simulink model "ng_pv_dynamic_dbus_p_1_sm_ng"  (Simulink 8.8)
settings: Solver=ode4  StartTime=0.0  StopTime=inf  FixedStep=0.000125  RelTol=1e-3  EnableMultiTasking=on
PreLoadFcn:
  | Ts=125e-6;Core_Num = 0; np=1; nq=1; Vmin=.9;
PostLoadFcn:
  | Ts=125e-6;Core_Num = 0; np=1; nq=1; Vmin=.9;
InitFcn:
  | Ts=125e-6;Core_Num = 0; np=1; nq=1; Vmin=.9;
undefined symbols (not defined in the file or in its folder): another_event_name, DiscIntNeverNeededParam, I, j, Left, my_event_name, Right, type, V, X
libraries: powerlib x316, simulink_extras x78, powerlib_meascontrol x47, ssn_lib x9, opal_lib x5, powerlib_extras x3, simulink x3, artemis x1, rtio_opalrt_ml605ex1 x1, rtlab x1, rtio_spectracom x1
(part 2 of 11)

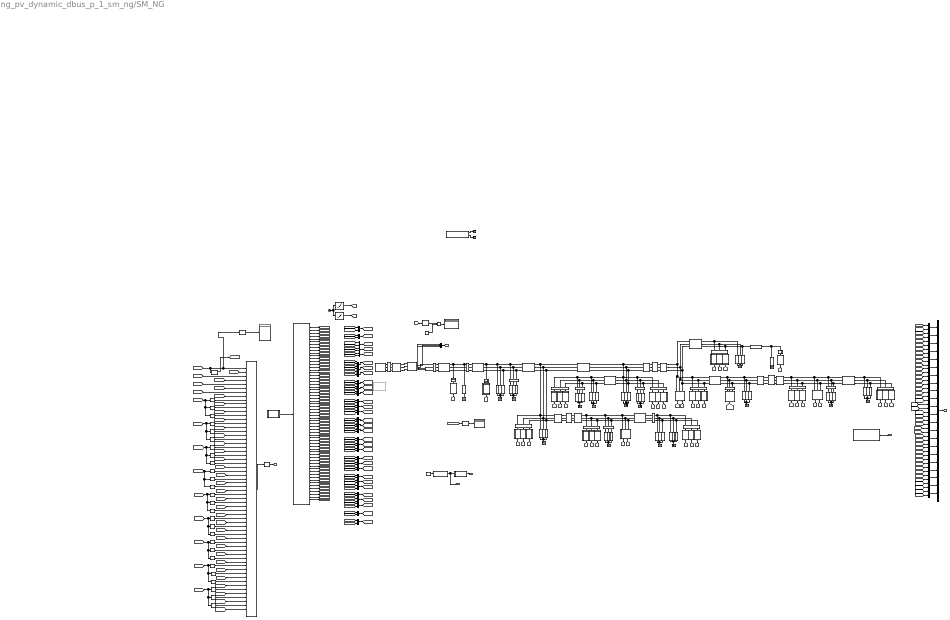
== system ng_pv_dynamic_dbus_p_1_sm_ng/SM_NG ==
  Bus Creator : BusCreator  Inputs=22
  Clock1 : Clock
  Constant : Constant  Value=13800/sqrt(3)
  Constant8 : Constant
  Demux1 : Demux  Outputs=62
  Display : Display
  Display1 : Display
  Divide : Product  Inputs=*/
  Dynamic Load BCDC1 : Subsystem
      mask Display:
      | plot(-45,-45,45,45,[0,9,18,24,29,30,29,24,18,9,0,-9,-18,-24,-29,-30,-29,-24,-18,-9,0]*.9,[30,29,24,18,9,0,-9,-18,-24,-29,-30,-29,-24,-18,-9,0,9,18,24,29,30]*.9)
      | plot([0,0,10,0,-10,0]*1.1,[15,-5,-5,-15,-5,-5]*1.1)
  Dynamic Load BCDC2 : Subsystem
      mask Display:
      | plot(-45,-45,45,45,[0,9,18,24,29,30,29,24,18,9,0,-9,-18,-24,-29,-30,-29,-24,-18,-9,0]*.9,[30,29,24,18,9,0,-9,-18,-24,-29,-30,-29,-24,-18,-9,0,9,18,24,29,30]*.9)
      | plot([0,0,10,0,-10,0]*1.1,[15,-5,-5,-15,-5,-5]*1.1)
  Dynamic Load BCDC3 : Subsystem
      mask Display:
      | plot(-45,-45,45,45,[0,9,18,24,29,30,29,24,18,9,0,-9,-18,-24,-29,-30,-29,-24,-18,-9,0]*.9,[30,29,24,18,9,0,-9,-18,-24,-29,-30,-29,-24,-18,-9,0,9,18,24,29,30]*.9)
      | plot([0,0,10,0,-10,0]*1.1,[15,-5,-5,-15,-5,-5]*1.1)
  Dynamic load measurement output1 : Display
  Ground{3,8,10,14,16,40,42..48,55,68..69} (16 alike) : powerlib/Elements/Ground  LConnTagsString=a
  IED1 : powerlib/Measurements/Three-Phase V-I Measurement  VoltageMeasurement=phase-to-ground  SetLabelV=on  LabelV=V_IED1  Vpu=off  VpuLL=off  CurrentMeasurement=yes  SetLabelI=on  LabelI=I_IED1  Ipu=off  Pbase=100e6  Vbase=500e3  OutputType=Complex  PhasorSimulation=off  PSBequivalent=0
  IED10 : Subsystem
      mask Display: %
  IED11 : powerlib/Measurements/Three-Phase V-I Measurement  VoltageMeasurement=phase-to-ground  SetLabelV=on  LabelV=V_IED11  Vpu=off  VpuLL=off  CurrentMeasurement=yes  SetLabelI=on  LabelI=I_IED11  Ipu=off  Pbase=100e6  Vbase=500e3  OutputType=Complex  PhasorSimulation=off  PSBequivalent=0
  IED12 : powerlib/Measurements/Three-Phase V-I Measurement  VoltageMeasurement=phase-to-ground  SetLabelV=on  LabelV=V_IED12  Vpu=off  VpuLL=off  CurrentMeasurement=yes  SetLabelI=on  LabelI=I_IED12  Ipu=off  Pbase=100e6  Vbase=500e3  OutputType=Complex  PhasorSimulation=off  PSBequivalent=0
  IED12A : powerlib/Measurements/Three-Phase V-I Measurement  VoltageMeasurement=phase-to-ground  SetLabelV=on  LabelV=V_IED12A  Vpu=off  VpuLL=off  CurrentMeasurement=yes  SetLabelI=on  LabelI=I_IED12A  Ipu=off  Pbase=100e6  Vbase=500e3  OutputType=Complex  PhasorSimulation=off  PSBequivalent=0
  IED13 : powerlib/Measurements/Three-Phase V-I Measurement  VoltageMeasurement=phase-to-ground  SetLabelV=on  LabelV=V_IED13  Vpu=off  VpuLL=off  CurrentMeasurement=yes  SetLabelI=on  LabelI=I_IED13  Ipu=off  Pbase=100e6  Vbase=500e3  OutputType=Complex  PhasorSimulation=off  PSBequivalent=0
  IED13A : powerlib/Measurements/Three-Phase V-I Measurement  VoltageMeasurement=phase-to-ground  SetLabelV=on  LabelV=V_IED13A  Vpu=off  VpuLL=off  CurrentMeasurement=yes  SetLabelI=on  LabelI=I_IED13A  Ipu=off  Pbase=100e6  Vbase=500e3  OutputType=Complex  PhasorSimulation=off  PSBequivalent=0
  IED14 : powerlib/Measurements/Three-Phase V-I Measurement  VoltageMeasurement=phase-to-ground  SetLabelV=on  LabelV=V_IED14  Vpu=off  VpuLL=off  CurrentMeasurement=yes  SetLabelI=on  LabelI=I_IED14  Ipu=off  Pbase=100e6  Vbase=500e3  OutputType=Complex  PhasorSimulation=off  PSBequivalent=0
  IED14A : Subsystem
      mask Display: %
  IED15 : powerlib/Measurements/Three-Phase V-I Measurement  VoltageMeasurement=phase-to-ground  SetLabelV=on  LabelV=V_IED15  Vpu=off  VpuLL=off  CurrentMeasurement=yes  SetLabelI=on  LabelI=I_IED15  Ipu=off  Pbase=100e6  Vbase=500e3  OutputType=Complex  PhasorSimulation=off  PSBequivalent=0
  IED2 : powerlib/Measurements/Three-Phase V-I Measurement  VoltageMeasurement=phase-to-ground  SetLabelV=on  LabelV=V_IED2  Vpu=off  VpuLL=off  CurrentMeasurement=yes  SetLabelI=on  LabelI=I_IED2  Ipu=off  Pbase=100e6  Vbase=500e3  OutputType=Complex  PhasorSimulation=off  PSBequivalent=0
  IED2A : powerlib/Measurements/Three-Phase V-I Measurement  VoltageMeasurement=phase-to-ground  SetLabelV=on  LabelV=V_IED2A  Vpu=off  VpuLL=off  CurrentMeasurement=yes  SetLabelI=on  LabelI=I_IED2A  Ipu=off  Pbase=100e6  Vbase=500e3  OutputType=Complex  PhasorSimulation=off  PSBequivalent=0
  IED3 : powerlib/Measurements/Three-Phase V-I Measurement  VoltageMeasurement=phase-to-ground  SetLabelV=on  LabelV=V_IED3  Vpu=off  VpuLL=off  CurrentMeasurement=yes  SetLabelI=on  LabelI=I_IED3  Ipu=off  Pbase=100e6  Vbase=500e3  OutputType=Complex  PhasorSimulation=off  PSBequivalent=0
  IED4 : powerlib/Measurements/Three-Phase V-I Measurement  VoltageMeasurement=phase-to-ground  SetLabelV=on  LabelV=V_IED4  Vpu=off  VpuLL=off  CurrentMeasurement=yes  SetLabelI=on  LabelI=I_IED4  Ipu=off  Pbase=100e6  Vbase=500e3  OutputType=Complex  PhasorSimulation=off  PSBequivalent=0
  IED5 : powerlib/Measurements/Three-Phase V-I Measurement  VoltageMeasurement=phase-to-ground  SetLabelV=on  LabelV=V_IED5  Vpu=off  VpuLL=off  CurrentMeasurement=yes  SetLabelI=on  LabelI=I_IED5  Ipu=off  Pbase=100e6  Vbase=500e3  OutputType=Complex  PhasorSimulation=off  PSBequivalent=0
  IED5A : powerlib/Measurements/Three-Phase V-I Measurement  VoltageMeasurement=phase-to-ground  SetLabelV=on  LabelV=V_IED5A  Vpu=off  VpuLL=off  CurrentMeasurement=yes  SetLabelI=on  LabelI=I_IED5A  Ipu=off  Pbase=100e6  Vbase=500e3  OutputType=Complex  PhasorSimulation=off  PSBequivalent=0
  IED6 : powerlib/Measurements/Three-Phase V-I Measurement  VoltageMeasurement=phase-to-ground  SetLabelV=on  LabelV=V_IED6  Vpu=off  VpuLL=off  CurrentMeasurement=yes  SetLabelI=on  LabelI=I_IED6  Ipu=off  Pbase=100e6  Vbase=500e3  OutputType=Complex  PhasorSimulation=off  PSBequivalent=0
  IED6A : powerlib/Measurements/Three-Phase V-I Measurement  VoltageMeasurement=phase-to-ground  SetLabelV=on  LabelV=V_IED6A  Vpu=off  VpuLL=off  CurrentMeasurement=yes  SetLabelI=on  LabelI=I_IED6A  Ipu=off  Pbase=100e6  Vbase=500e3  OutputType=Complex  PhasorSimulation=off  PSBequivalent=0
  IED7 : powerlib/Measurements/Three-Phase V-I Measurement  VoltageMeasurement=phase-to-ground  SetLabelV=on  LabelV=V_IED7  Vpu=off  VpuLL=off  CurrentMeasurement=yes  SetLabelI=on  LabelI=I_IED7  Ipu=off  Pbase=100e6  Vbase=500e3  OutputType=Complex  PhasorSimulation=off  PSBequivalent=0
  IED7A : Subsystem
      mask Display: %
  IED8 : powerlib/Measurements/Three-Phase V-I Measurement  VoltageMeasurement=phase-to-ground  SetLabelV=on  LabelV=V_IED8  Vpu=off  VpuLL=off  CurrentMeasurement=yes  SetLabelI=on  LabelI=I_IED8  Ipu=off  Pbase=100e6  Vbase=500e3  OutputType=Complex  PhasorSimulation=off  PSBequivalent=0
  IED9 : powerlib/Measurements/Three-Phase V-I Measurement  VoltageMeasurement=phase-to-ground  SetLabelV=on  LabelV=V_IED9  Vpu=off  VpuLL=off  CurrentMeasurement=yes  SetLabelI=on  LabelI=I_IED9  Ipu=off  Pbase=100e6  Vbase=500e3  OutputType=Complex  PhasorSimulation=off  PSBequivalent=0
  Line1132 : powerlib/Elements/Three-Phase PI Section Line  LConnTagsString=a|b|c  RConnTagsString=A|B|C  Frequency=60  Resistances=[0.071333 1.193903]  Inductances=[0.000315639 0.00352311]  Capacitances=[1.83433E-07 2.8E-13]  Length=0.067056
  Line3 : powerlib/Elements/Three-Phase PI Section Line  Commented=on  LConnTagsString=a|b|c  RConnTagsString=A|B|C  Frequency=60  Resistances=[0.0339 0.0293]  Inductances=[1.0783 1.0436]/(2*pi()*60)  Capacitances=[1E-16 1E-16]  Length=1
  Line369 : powerlib/Elements/Three-Phase PI Section Line  LConnTagsString=a|b|c  RConnTagsString=A|B|C  Frequency=60  Resistances=[2.631377E-01 0.6660566]  Inductances=[0.001030059 0.003789301]  Capacitances=[1.0e-16 1.0e-16]  Length=5.012741
  Line405A : powerlib/Elements/Three-Phase PI Section Line  LConnTagsString=a|b|c  RConnTagsString=A|B|C  Frequency=60  Resistances=[0.1736172 0.5584416]  Inductances=[0.001078896 0.003407176]  Capacitances=[1E-16 1E-16]  Length=0.7351776/2
  Line405B : powerlib/Elements/Three-Phase PI Section Line  LConnTagsString=a|b|c  RConnTagsString=A|B|C  Frequency=60  Resistances=[0.1736172 0.5584416]  Inductances=[0.001078896 0.003407176]  Capacitances=[1E-16 1E-16]  Length=0.7351776/2
  Line425 : powerlib/Elements/Three-Phase PI Section Line  LConnTagsString=a|b|c  RConnTagsString=A|B|C  Frequency=60  Resistances=[0.2736189 0.6685028]  Inductances=[0.001062159 0.003997129]  Capacitances=[1.0e-16 1.0e-16]  Length=2.185111
  Line489 : powerlib/Elements/Three-Phase PI Section Line  LConnTagsString=a|b|c  RConnTagsString=A|B|C  Frequency=60  Resistances=[0.118123 0.5162969]  Inductances=[0.000848017 0.003875996]  Capacitances=[1.0e-16 1.0e-16]  Length=0.2593848
  Line491 : powerlib/Elements/Three-Phase PI Section Line  LConnTagsString=a|b|c  RConnTagsString=A|B|C  Frequency=60  Resistances=[0.1181207 0.5161311]  Inductances=[0.00084801 0.003875749]  Capacitances=[1.0e-16 1.0e-16]  Length=3.555187
  Line614 : powerlib/Elements/Pi Section Line  LConnTagsString=__new0  RConnTagsString=__new0  Frequency=60  Resistance=1.074502  Inductance=0.001854886  Capacitance=1e-18  Length=1.515161  PiSections=1  Measurements=None
      settings: AttributesFormatString=\n
  Line687 : powerlib/Elements/Three-Phase PI Section Line  LConnTagsString=a|b|c  RConnTagsString=A|B|C  Frequency=60  Resistances=[1.671830E-01 0.5617232]  Inductances=[0.000886022 0.00391557]  Capacitances=[1.0e-16 1.0e-16]  Length=0.745236
  Line718A : powerlib/Elements/Three-Phase PI Section Line  LConnTagsString=a|b|c  RConnTagsString=A|B|C  Frequency=60  Resistances=[1.670246E-01 0.5628342]  Inductances=[0.000882962 0.00392461]  Capacitances=[1.0e-16 1.0e-16]  Length=1.407871/2
  Line718B : powerlib/Elements/Three-Phase PI Section Line  LConnTagsString=a|b|c  RConnTagsString=A|B|C  Frequency=60  Resistances=[1.670246E-01 0.5628342]  Inductances=[0.000882962 0.00392461]  Capacitances=[1.0e-16 1.0e-16]  Length=1.407871/2
  Line775A : powerlib/Elements/Three-Phase PI Section Line  LConnTagsString=a|b|c  RConnTagsString=A|B|C  Frequency=60  Resistances=[0.167158 0.5649899]  Inductances=[0.000879297 0.003911286]  Capacitances=[1.0e-16 1.0e-16]  Length=1.061314/2
  Line775B : powerlib/Elements/Three-Phase PI Section Line  LConnTagsString=a|b|c  RConnTagsString=A|B|C  Frequency=60  Resistances=[0.167158 0.5649899]  Inductances=[0.000879297 0.003911286]  Capacitances=[1.0e-16 1.0e-16]  Length=1.061314/2
  Line777 : powerlib/Elements/Three-Phase PI Section Line  LConnTagsString=a|b|c  RConnTagsString=A|B|C  Frequency=60  Resistances=[0.1732583 0.5348146]  Inductances=[0.000986024 0.00348674]  Capacitances=[1E-16 1E-16]  Length=0.6230112
  Line809 : powerlib/Elements/Three-Phase PI Section Line  LConnTagsString=a|b|c  RConnTagsString=A|B|C  Frequency=60  Resistances=[0.2709616 0.6137313]  Inductances=[0.00111084 0.00345815]  Capacitances=[1.0e-16 1.0e-16]  Length=2.52923
  Line937 : powerlib/Elements/Three-Phase PI Section Line  LConnTagsString=a|b|c  RConnTagsString=A|B|C  Frequency=60  Resistances=[0.1181214 0.5162814]  Inductances=[0.000848012 0.003875967]  Capacitances=[1.0e-16 1.0e-16]  Length=3.339389
  Mux{,1..4,6..53} (53 alike) : Mux  Inputs=2
  Mux5 : Mux  Inputs=62
  Mux54 : Mux  Inputs=3
  OpCtrl ML605EX1 : rtio_opalrt_ml605ex1/OpCtrl ML605EX1  CtrlName='ML605EX1 Ctrl'  boardid=0  BitstreamFilename=ML605_2-EX-0029-2_2_6_61-32Aio_32DioSelectable-01-01.bin  numconfig=-1  mode=Master  externalClock=off  decimRtsi=0  calibIO=off  SampleTime=0  loadinport=-1
  OpMonitor : rtlab/Monitoring/OpMonitor  compute_time=off  real_step=off  idle_time=off  nb_overruns=on  user_time=off  user_name=my_event_name,another_event_name
  PLL (3ph)2 : powerlib_meascontrol/PLL/PLL (3ph)  Fmin=45  Par_Init=[0, 60]  ParK=[180, 3200, 1]  TcD=1e-4  MaxRateChangeFreq=12  FilterCutOffFreq=25  Ts=0  AGC=on
  PV11 : Subsystem
      mask Display:
      | plot(.2*[0 3.5 5 2 0], .2*[1 1 4.5 4.5 1])
      | plot(.2*[1.7 3.5], .2*[1 4.5])
      | plot(.2*[1.1 4.3], .2*[3 3])
      | plot(.2*[.6 3.9], .2*[2 2])
      | plot(.2*[1.7 4.7], .2*[3.9 3.9])
  RMS : powerlib_meascontrol/Measurements/RMS  TrueRMS=on  Freq=60  RMSInit=120  Ts=0
  RMS2 : powerlib_meascontrol/Measurements/RMS  TrueRMS=on  Freq=60  RMSInit=480  Ts=Ts
  RMS28 : powerlib_meascontrol/Measurements/RMS  TrueRMS=on  Freq=60  RMSInit=480  Ts=Ts
  RMS3 : powerlib_meascontrol/Measurements/RMS  TrueRMS=on  Freq=60  RMSInit=13.8e3/sqrt(3)  Ts=Ts
  Real Power : Lookup_n-D  NumberOfTableDimensions=1  BreakpointsForDimension1=|  Table=|  ExtrapMethod=Clip  RndMeth=Simplest  InputSameDT=on
      BreakpointsForDimension1=|
      | [0
      | 900
      | 1800
      | 2700
      | 3600
      | 4500
      | 5400
      | 6300
      | 7200
      | 8100
      | 9000
      | 9900
      | 10800
      | 11700
      | 12600
      | 13500
      | 14400
      | 15300
      | 16200
      | 17100
      | 18000
      | 18900
      | 19800
      | 20700
      | 21600
      | ]
      Table=|
      | [0.386455785
      | 0.35306969
      | 0.331026162
      | 0.30769857
      | 0.305344452
      | 0.311122953
      | 0.342154931
      | 0.435946389
      | 0.489666766
      | 0.534959927
      | 0.558308136
      | 0.579659692
      | 0.643062563
      | 0.611273703
      | 0.64816703
      | 0.579694179
      | 0.56936906
      | 0.534896062
      | 0.526366773
      | 0.521782301
      | 0.502521358
      | 0.511800972
      | 0.405864397
      | 0.369267928
      | 0.34401424]
  Real Power1 : Lookup_n-D  NumberOfTableDimensions=1  BreakpointsForDimension1=|  Table=|  ExtrapMethod=Clip  RndMeth=Simplest  InputSameDT=on
      BreakpointsForDimension1=|
      | [0
      | 900
      | 1800
      | 2700
      | 3600
      | 4500
      | 5400
      | 6300
      | 7200
      | 8100
      | 9000
      | 9900
      | 10800
      | 11700
      | 12600
      | 13500
      | 14400
      | 15300
      | 16200
      | 17100
      | 18000
      | 18900
      | 19800
      | 20700
      | 21600
      | ]
      Table=|
      | [0.386455785
      | 0.35306969
      | 0.331026162
      | 0.30769857
      | 0.305344452
      | 0.311122953
      | 0.342154931
      | 0.435946389
      | 0.489666766
      | 0.534959927
      | 0.558308136
      | 0.579659692
      | 0.643062563
      | 0.611273703
      | 0.64816703
      | 0.579694179
      | 0.56936906
      | 0.534896062
      | 0.526366773
      | 0.521782301
      | 0.502521358
      | 0.511800972
      | 0.405864397
      | 0.369267928
      | 0.34401424]
  SSN Interface Block (3ph) : ssn_lib/SSN Interface Block (3ph)  nb_phase=3  nb_port=2  p1_type=I-type(Left)  p2_type=I-type(Right)  p3_type=V-type(Left)  p4_type=V-type(Left)  p5_type=V-type(Left)  p6_type=V-type(Left)  p7_type=V-type(Left)  p8_type=V-type(Left)  p9_type=V-type(Left)  p10_type=V-type(Left)  p11_type=V-type(Left)  p12_type=V-type(Left)  p13_type=V-type(Left)  p14_type=V-type(Left)  p15_type=V-type(Left)  p16_type=V-type(Left)  I_port_shunt_resistance=1e9
  SSN Interface Block (3ph)1 : ssn_lib/SSN Interface Block (3ph)  nb_phase=3  nb_port=2  p1_type=I-type(Left)  p2_type=I-type(Right)  p3_type=V-type(Left)  p4_type=V-type(Left)  p5_type=V-type(Left)  p6_type=V-type(Left)  p7_type=V-type(Left)  p8_type=V-type(Left)  p9_type=V-type(Left)  p10_type=V-type(Left)  p11_type=V-type(Left)  p12_type=V-type(Left)  p13_type=V-type(Left)  p14_type=V-type(Left)  p15_type=V-type(Left)  p16_type=V-type(Left)  I_port_shunt_resistance=1e9
  SSN Interface Block (3ph)2 : ssn_lib/SSN Interface Block (3ph)  nb_phase=3  nb_port=2  p1_type=I-type(Left)  p2_type=I-type(Right)  p3_type=V-type(Left)  p4_type=V-type(Left)  p5_type=V-type(Left)  p6_type=V-type(Left)  p7_type=V-type(Left)  p8_type=V-type(Left)  p9_type=V-type(Left)  p10_type=V-type(Left)  p11_type=V-type(Left)  p12_type=V-type(Left)  p13_type=V-type(Left)  p14_type=V-type(Left)  p15_type=V-type(Left)  p16_type=V-type(Left)  I_port_shunt_resistance=1e9
  Selector{7,10,13,16,19,22,25,28,31} (9 alike) : Selector  InputPortWidth=3  IndexOptions=Index vector (dialog)  Indices=[2]  OutputSizes=1
  Selector{8,11,14,17,20,23,26,29,32} (9 alike) : Selector  InputPortWidth=3  IndexOptions=Index vector (dialog)  Indices=[3]  OutputSizes=1
  Selector{6,9,12,15,18,21,24,27,30} (9 alike) : Selector  InputPortWidth=3  IndexOptions=Index vector (dialog)  Indices=[1]  OutputSizes=1
  Series  Load100 : powerlib/Elements/Series RLC Load  LConnTagsString=a  RConnTagsString=__new0  NominalVoltage=7967.4337  NominalFrequency=60  ActivePower=95731.2873  InductivePower=45807.5351  CapacitivePower=0  Setx0=off  InitialVoltage=0  SetiL0=off  InitialCurrent=0  Measurements=None  LoadType=constant Z
  Series  Load22 : powerlib/Elements/Series RLC Load  LConnTagsString=a  RConnTagsString=__new0  NominalVoltage=7967.4337  NominalFrequency=60  ActivePower=331147.6000  InductivePower=210430.3000  CapacitivePower=0  Setx0=off  InitialVoltage=0  SetiL0=off  InitialCurrent=0  Measurements=None  LoadType=constant Z
  Series  Load23 : powerlib/Elements/Series RLC Load  LConnTagsString=a  RConnTagsString=__new0  NominalVoltage=7967.4337  NominalFrequency=60  ActivePower=241844.2000  InductivePower=147122.1000  CapacitivePower=0  Setx0=off  InitialVoltage=0  SetiL0=off  InitialCurrent=0  Measurements=None  LoadType=constant Z
  Series  Load24 : powerlib/Elements/Series RLC Load  LConnTagsString=a  RConnTagsString=__new0  NominalVoltage=7967.4337  NominalFrequency=60  ActivePower=195882.9000  InductivePower=92467.2000  CapacitivePower=0  Setx0=off  InitialVoltage=0  SetiL0=off  InitialCurrent=0  Measurements=None  LoadType=constant Z
  Series  Load28 : powerlib/Elements/Series RLC Load  LConnTagsString=a  RConnTagsString=__new0  NominalVoltage=7967.4337  NominalFrequency=60  ActivePower=4813.9386  InductivePower=3013.6069  CapacitivePower=0  Setx0=off  InitialVoltage=0  SetiL0=off  InitialCurrent=0  Measurements=None  LoadType=constant Z
  Series  Load{42,60,80..83,91..96} (12 alike) : powerlib/Elements/Series RLC Load  LConnTagsString=a  RConnTagsString=__new0  NominalVoltage=7970  NominalFrequency=60  ActivePower=0  InductivePower=0  CapacitivePower=600000/3  Setx0=off  InitialVoltage=0  SetiL0=off  InitialCurrent=0  Measurements=None  LoadType=constant Z
  Series  Load43 : powerlib/Elements/Series RLC Load  LConnTagsString=a  RConnTagsString=__new0  NominalVoltage=7967.4337  NominalFrequency=60  ActivePower=4551.0724  InductivePower=2264.2140  CapacitivePower=0  Setx0=off  InitialVoltage=0  SetiL0=off  InitialCurrent=0  Measurements=None  LoadType=constant Z
  Series  Load61 : powerlib/Elements/Series RLC Load  LConnTagsString=a  RConnTagsString=__new0  NominalVoltage=7967.4337  NominalFrequency=60  ActivePower=282693.5835  InductivePower=180806.3086  CapacitivePower=0  Setx0=off  InitialVoltage=0  SetiL0=off  InitialCurrent=0  Measurements=None  LoadType=constant Z
  Series  Load62 : powerlib/Elements/Series RLC Load  LConnTagsString=a  RConnTagsString=__new0  NominalVoltage=7967.4337  NominalFrequency=60  ActivePower=208215.9420  InductivePower=105579.1068  CapacitivePower=0  Setx0=off  InitialVoltage=0  SetiL0=off  InitialCurrent=0  Measurements=None  LoadType=constant Z
  Series  Load63 : powerlib/Elements/Series RLC Load  LConnTagsString=a  RConnTagsString=__new0  NominalVoltage=7967.4337  NominalFrequency=60  ActivePower=421137.8951  InductivePower=259530.0314  CapacitivePower=0  Setx0=off  InitialVoltage=0  SetiL0=off  InitialCurrent=0  Measurements=None  LoadType=constant Z
  Series  Load64 : powerlib/Elements/Series RLC Load  LConnTagsString=a  RConnTagsString=__new0  NominalVoltage=7967.4337  NominalFrequency=60  ActivePower=122799.6001  InductivePower=58366.8938  CapacitivePower=0  Setx0=off  InitialVoltage=0  SetiL0=off  InitialCurrent=0  Measurements=None  LoadType=constant Z
  Series  Load7 : powerlib/Elements/Series RLC Load  LConnTagsString=a  RConnTagsString=__new0  NominalVoltage=7967.4337  NominalFrequency=60  ActivePower=612731.0000  InductivePower=318097.6000  CapacitivePower=0  Setx0=off  InitialVoltage=0  SetiL0=off  InitialCurrent=0  Measurements=None  LoadType=constant Z
  Series  Load71 : powerlib/Elements/Series RLC Load  LConnTagsString=a  RConnTagsString=__new0  NominalVoltage=7967.4337  NominalFrequency=60  ActivePower=10751.6072  InductivePower=5034.6946  CapacitivePower=0  Setx0=off  InitialVoltage=0  SetiL0=off  InitialCurrent=0  Measurements=None  LoadType=constant Z
  Series  Load72 : powerlib/Elements/Series RLC Load  LConnTagsString=a  RConnTagsString=__new0  NominalVoltage=7967.4337  NominalFrequency=60  ActivePower=118772.0877  InductivePower=74481.4641  CapacitivePower=0  Setx0=off  InitialVoltage=0  SetiL0=off  InitialCurrent=0  Measurements=None  LoadType=constant Z
  Series  Load73 : powerlib/Elements/Series RLC Load  LConnTagsString=a  RConnTagsString=__new0  NominalVoltage=7967.4337  NominalFrequency=60  ActivePower=132738.7273  InductivePower=44254.9312  CapacitivePower=0  Setx0=off  InitialVoltage=0  SetiL0=off  InitialCurrent=0  Measurements=None  LoadType=constant Z
  Series  Load74 : powerlib/Elements/Series RLC Load  LConnTagsString=a  RConnTagsString=__new0  NominalVoltage=7967.4337  NominalFrequency=60  ActivePower=81396.3132  InductivePower=49692.8288  CapacitivePower=0  Setx0=off  InitialVoltage=0  SetiL0=off  InitialCurrent=0  Measurements=None  LoadType=constant Z
  Series  Load75 : powerlib/Elements/Series RLC Load  LConnTagsString=a  RConnTagsString=__new0  NominalVoltage=7967.4337  NominalFrequency=60  ActivePower=22321.0824  InductivePower=10622.5578  CapacitivePower=0  Setx0=off  InitialVoltage=0  SetiL0=off  InitialCurrent=0  Measurements=None  LoadType=constant Z
  Series  Load76 : powerlib/Elements/Series RLC Load  LConnTagsString=a  RConnTagsString=__new0  NominalVoltage=7967.4337  NominalFrequency=60  ActivePower=333509.6803  InductivePower=179550.2294  CapacitivePower=0  Setx0=off  InitialVoltage=0  SetiL0=off  InitialCurrent=0  Measurements=None  LoadType=constant Z
  Series  Load77 : powerlib/Elements/Series RLC Load  LConnTagsString=a  RConnTagsString=__new0  NominalVoltage=7967.4337  NominalFrequency=60  ActivePower=249017.5283  InductivePower=118318.2378  CapacitivePower=0  Setx0=off  InitialVoltage=0  SetiL0=off  InitialCurrent=0  Measurements=None  LoadType=constant Z
  Series  Load78 : powerlib/Elements/Series RLC Load  LConnTagsString=a  RConnTagsString=__new0  NominalVoltage=7967.4337  NominalFrequency=60  ActivePower=191185.4608  InductivePower=115039.6819  CapacitivePower=0  Setx0=off  InitialVoltage=0  SetiL0=off  InitialCurrent=0  Measurements=None  LoadType=constant Z
  Series  Load79 : powerlib/Elements/Series RLC Load  LConnTagsString=a  RConnTagsString=__new0  NominalVoltage=7967.4337  NominalFrequency=60  ActivePower=315752.0854  InductivePower=102715.4164  CapacitivePower=0  Setx0=off  InitialVoltage=0  SetiL0=off  InitialCurrent=0  Measurements=None  LoadType=constant Z
  Series  Load8 : powerlib/Elements/Series RLC Load  LConnTagsString=a  RConnTagsString=__new0  NominalVoltage=7967.4337  NominalFrequency=60  ActivePower=406958.6000  InductivePower=209692.6000  CapacitivePower=0  Setx0=off  InitialVoltage=0  SetiL0=off  InitialCurrent=0  Measurements=None  LoadType=constant Z
  Series  Load84 : powerlib/Elements/Series RLC Load  LConnTagsString=a  RConnTagsString=__new0  NominalVoltage=7970  NominalFrequency=60  ActivePower=0  InductivePower=0  CapacitivePower=1200000/3  Setx0=off  InitialVoltage=0  SetiL0=off  InitialCurrent=0  Measurements=None  LoadType=constant PQ
  Series  Load85 : powerlib/Elements/Series RLC Load  LConnTagsString=a  RConnTagsString=__new0  NominalVoltage=7970  NominalFrequency=60  ActivePower=0  InductivePower=0  CapacitivePower=1200000/3  Setx0=off  InitialVoltage=0  SetiL0=off  InitialCurrent=0  Measurements=None  LoadType=constant PQ
  Series  Load86 : powerlib/Elements/Series RLC Load  LConnTagsString=a  RConnTagsString=__new0  NominalVoltage=7967.4337  NominalFrequency=60  ActivePower=108322.5585  InductivePower=62208.1391  CapacitivePower=0  Setx0=off  InitialVoltage=0  SetiL0=off  InitialCurrent=0  Measurements=None  LoadType=constant Z
  Series  Load87 : powerlib/Elements/Series RLC Load  LConnTagsString=a  RConnTagsString=__new0  NominalVoltage=7970  NominalFrequency=60  ActivePower=0  InductivePower=0  CapacitivePower=1200000/3  Setx0=off  InitialVoltage=0  SetiL0=off  InitialCurrent=0  Measurements=None  LoadType=constant PQ
  Series  Load88 : powerlib/Elements/Series RLC Load  LConnTagsString=a  RConnTagsString=__new0  NominalVoltage=7970  NominalFrequency=60  ActivePower=0  InductivePower=0  CapacitivePower=900000/3  Setx0=off  InitialVoltage=0  SetiL0=off  InitialCurrent=0  Measurements=None  LoadType=constant Z
  Series  Load89 : powerlib/Elements/Series RLC Load  LConnTagsString=a  RConnTagsString=__new0  NominalVoltage=7970  NominalFrequency=60  ActivePower=0  InductivePower=0  CapacitivePower=900000/3  Setx0=off  InitialVoltage=0  SetiL0=off  InitialCurrent=0  Measurements=None  LoadType=constant Z
  Series  Load9 : powerlib/Elements/Series RLC Load  LConnTagsString=a  RConnTagsString=__new0  NominalVoltage=7967.4337  NominalFrequency=60  ActivePower=419138.0000  InductivePower=167037.2000  CapacitivePower=0  Setx0=off  InitialVoltage=0  SetiL0=off  InitialCurrent=0  Measurements=None  LoadType=constant Z
  Series  Load90 : powerlib/Elements/Series RLC Load  LConnTagsString=a  RConnTagsString=__new0  NominalVoltage=7970  NominalFrequency=60  ActivePower=0  InductivePower=0  CapacitivePower=900000/3  Setx0=off  InitialVoltage=0  SetiL0=off  InitialCurrent=0  Measurements=None  LoadType=constant Z
  Series  Load97 : powerlib/Elements/Series RLC Load  LConnTagsString=a  RConnTagsString=__new0  NominalVoltage=7967.4337  NominalFrequency=60  ActivePower=91473.9797  InductivePower=41476.5707  CapacitivePower=0  Setx0=off  InitialVoltage=0  SetiL0=off  InitialCurrent=0  Measurements=None  LoadType=constant Z
  Series  Load98 : powerlib/Elements/Series RLC Load  LConnTagsString=a  RConnTagsString=__new0  NominalVoltage=7967.4337  NominalFrequency=60  ActivePower=276895.7686  InductivePower=217638.0421  CapacitivePower=0  Setx0=off  InitialVoltage=0  SetiL0=off  InitialCurrent=0  Measurements=None  LoadType=constant Z
  Series  Load99 : powerlib/Elements/Series RLC Load  LConnTagsString=a  RConnTagsString=__new0  NominalVoltage=7967.4337  NominalFrequency=60  ActivePower=181389.9148  InductivePower=112840.1531  CapacitivePower=0  Setx0=off  InitialVoltage=0  SetiL0=off  InitialCurrent=0  Measurements=None  LoadType=constant Z
  Single-Phase Dynamic Load30 : Subsystem  DialogController=POWERSYS.PowerSysDialog  mask(Single-Phase Dynamic Load){NominalVoltage=|, ActiveReactivePowers=[-27219.200 432.132], PositiveSequence=[1 0], ExternalControl=on, NpNq=[np nq], TimeConstants=[0  0  0  0], MinimumVoltage=Vmin, LoadFlowParameters=[4,0,0,0,0]}
      mask NominalVoltage=|
      | [7967.43
      |  60]
      mask prompts: NominalVoltage "Nominal voltage and frequency  [Vn(Vrms) fn(Hz)]:"; ActiveReactivePowers "Active and reactive power at initial voltage [Po(W) Qo(var)]:"; PositiveSequence "Initial voltage Vo [Mag(pu) Phase (deg.)]:"; ExternalControl "External control of PQ"; NpNq "Parameters [ np  nq ]:"; TimeConstants "Time constants [Tp1 Tp2 Tq1 Tq2]  (s):"; MinimumVoltage "Minimum voltage Vmin (pu):"; LoadFlowParameters "Load Flow parameters"
      mask help:
      | Implements a single-phase dynamic load. Active  power P and reactive
      | power Q absorbed by the load vary as function of voltage V  according to the
      | following equations:
      |
      |   If V>Vmin, P and Q vary as follows:
      |        P = Po * (V/Vo)^np * (1+Tp1.s)/(1+Tp2.s)
      |        Q = Qo * (V/Vo)^nq * (1+Tq1.s)/(1+Tq2.s)
      |   if V<Vmin
      |      Same equations with np=nq=2 (constant impedance load)
      mask init:
      | Vmin=.1;
      | 
      | Vnom=7967.43; 
      | fnom=60;
      | P0=-27219.200;
      | Q0=432.132;
      | Mag_V0=1; 
      | Pha_V0=0;
      | V0_d=1;
      | V0_q=Mag_V0*sin(Pha_V0*pi/180);
      | np=1;
      | nq=1;
      | Tp1=0; 
      | Tp2=0; 
      | Tq1=0; 
      | Tq2=0;
      | Vbase=Vnom/sqrt(3)*sqrt(2);
      | % initial value of positive-sequence current I1
      | I1_init=(P0-j*Q0)/((V0_d-j*V0_q)*Vnom)/sqrt(3)*sqrt(2);
      | Mag_ia=abs(I1_init);
      | Phase_ia=angle(I1_init)*180/pi;
      | %
      | a=exp(j*2*pi/3);
      | power_initmask();
      mask Help: helpview(psbhelp)
      mask Callback ExternalControl: powericon('ThreePhaseDynamicLoadCback',gcb);
      mask Display:
      | plot(.2*[0 3.5 5 2 0], .2*[1 1 4.5 4.5 1])
      | 
      | plot(.2*[1.7 3.5], .2*[1 4.5])
      | 
      | plot(.2*[1.1 4.3], .2*[3 3])
      | 
      | plot(.2*[.6 3.9], .2*[2 2])
      | 
      | plot(.2*[1.7 4.7], .2*[3.9 3.9])
  Single-Phase Dynamic Load32 : Subsystem  DialogController=POWERSYS.PowerSysDialog  mask(Single-Phase Dynamic Load){NominalVoltage=|, ActiveReactivePowers=|, PositiveSequence=[1 0], ExternalControl=on, NpNq=[np nq], TimeConstants=[0  0  0  0], MinimumVoltage=Vmin, LoadFlowParameters=[4,0,0,0,0]}
      mask NominalVoltage=|
      | [7967.43
      | 60]
      mask ActiveReactivePowers=|
      | [-277874.000
      | -40319.906]
      mask prompts: NominalVoltage "Nominal voltage and frequency  [Vn(Vrms) fn(Hz)]:"; ActiveReactivePowers "Active and reactive power at initial voltage [Po(W) Qo(var)]:"; PositiveSequence "Initial voltage Vo [Mag(pu) Phase (deg.)]:"; ExternalControl "External control of PQ"; NpNq "Parameters [ np  nq ]:"; TimeConstants "Time constants [Tp1 Tp2 Tq1 Tq2]  (s):"; MinimumVoltage "Minimum voltage Vmin (pu):"; LoadFlowParameters "Load Flow parameters"
      mask help:
      | Implements a single-phase dynamic load. Active  power P and reactive
      | power Q absorbed by the load vary as function of voltage V  according to the
      | following equations:
      |
      |   If V>Vmin, P and Q vary as follows:
      |        P = Po * (V/Vo)^np * (1+Tp1.s)/(1+Tp2.s)
      |        Q = Qo * (V/Vo)^nq * (1+Tq1.s)/(1+Tq2.s)
      |   if V<Vmin
      |      Same equations with np=nq=2 (constant impedance load)
      mask init:
      | block = gcb;
      | Ts = 50e-6;
      | %
      | Vnom=NominalVoltage(1); 
      | fnom=NominalVoltage(2);
      | P0=ActiveReactivePowers(1);
      | Q0=ActiveReactivePowers(2);
      | Mag_V0=PositiveSequence(1); 
      | Pha_V0=PositiveSequence(2);
      | V0_d=Mag_V0*cos(Pha_V0*pi/180);
      | V0_q=Mag_V0*sin(Pha_V0*pi/180);
      | np=NpNq(1);
      | nq=NpNq(2);
      | Tp1=TimeConstants(1); 
      | Tp2=TimeConstants(2); 
      | Tq1=TimeConstants(3); 
      | Tq2=TimeConstants(4);
      | Vbase=Vnom/sqrt(3)*sqrt(2);
      | % initial value of positive-sequence current I1
      | I1_init=(P0-j*Q0)/((V0_d-j*V0_q)*Vnom)/sqrt(3)*sqrt(2);
      | Mag_ia=abs(I1_init);
      | Phase_ia=angle(I1_init)*180/pi;
      | %
      | Vmin=MinimumVoltage;
      | PQext=ExternalControl;
      | a=exp(j*2*pi/3);
      | power_initmask();
      mask Help: helpview(psbhelp)
      mask Callback ExternalControl: powericon('ThreePhaseDynamicLoadCback',gcb);
      mask Display:
      | plot(.2*[0 3.5 5 2 0], .2*[1 1 4.5 4.5 1])
      | plot(.2*[1.7 3.5], .2*[1 4.5])
      | plot(.2*[1.1 4.3], .2*[3 3])
      | plot(.2*[.6 3.9], .2*[2 2])
      | plot(.2*[1.7 4.7], .2*[3.9 3.9])
  Single-Phase Dynamic Load33 : Subsystem  DialogController=POWERSYS.PowerSysDialog  mask(Single-Phase Dynamic Load){NominalVoltage=|, ActiveReactivePowers=|, PositiveSequence=[1 0], ExternalControl=on, NpNq=[np nq], TimeConstants=[0  0  0  0], MinimumVoltage=Vmin, LoadFlowParameters=[4,0,0,0,0]}
      mask NominalVoltage=|
      | [7967.43
      | 60]
      mask ActiveReactivePowers=|
      | [-127775.000
      | 18152.596]
      mask prompts: NominalVoltage "Nominal voltage and frequency  [Vn(Vrms) fn(Hz)]:"; ActiveReactivePowers "Active and reactive power at initial voltage [Po(W) Qo(var)]:"; PositiveSequence "Initial voltage Vo [Mag(pu) Phase (deg.)]:"; ExternalControl "External control of PQ"; NpNq "Parameters [ np  nq ]:"; TimeConstants "Time constants [Tp1 Tp2 Tq1 Tq2]  (s):"; MinimumVoltage "Minimum voltage Vmin (pu):"; LoadFlowParameters "Load Flow parameters"
      mask help:
      | Implements a single-phase dynamic load. Active  power P and reactive
      | power Q absorbed by the load vary as function of voltage V  according to the
      | following equations:
      |
      |   If V>Vmin, P and Q vary as follows:
      |        P = Po * (V/Vo)^np * (1+Tp1.s)/(1+Tp2.s)
      |        Q = Qo * (V/Vo)^nq * (1+Tq1.s)/(1+Tq2.s)
      |   if V<Vmin
      |      Same equations with np=nq=2 (constant impedance load)
      mask init: same as ng_pv_dynamic_dbus_p_1_sm_ng/SM_NG/Single-Phase Dynamic Load32
      mask Help: helpview(psbhelp)
      mask Callback ExternalControl: powericon('ThreePhaseDynamicLoadCback',gcb);
      mask Display:
      | plot(.2*[0 3.5 5 2 0], .2*[1 1 4.5 4.5 1])
      | plot(.2*[1.7 3.5], .2*[1 4.5])
      | plot(.2*[1.1 4.3], .2*[3 3])
      | plot(.2*[.6 3.9], .2*[2 2])
      | plot(.2*[1.7 4.7], .2*[3.9 3.9])
  Single-Phase Dynamic Load34 : Subsystem  DialogController=POWERSYS.PowerSysDialog  mask(Single-Phase Dynamic Load){NominalVoltage=|, ActiveReactivePowers=[-26871.400 3823.801], PositiveSequence=[1 0], ExternalControl=on, NpNq=[np nq], TimeConstants=[0  0  0  0], MinimumVoltage=Vmin, LoadFlowParameters=[4,0,0,0,0]}
      mask NominalVoltage=|
      | [ 7967.43
      | 60 ]
      mask prompts: NominalVoltage "Nominal voltage and frequency  [Vn(Vrms) fn(Hz)]:"; ActiveReactivePowers "Active and reactive power at initial voltage [Po(W) Qo(var)]:"; PositiveSequence "Initial voltage Vo [Mag(pu) Phase (deg.)]:"; ExternalControl "External control of PQ"; NpNq "Parameters [ np  nq ]:"; TimeConstants "Time constants [Tp1 Tp2 Tq1 Tq2]  (s):"; MinimumVoltage "Minimum voltage Vmin (pu):"; LoadFlowParameters "Load Flow parameters"
      mask help:
      | Implements a single-phase dynamic load. Active  power P and reactive
      | power Q absorbed by the load vary as function of voltage V  according to the
      | following equations:
      |
      |   If V>Vmin, P and Q vary as follows:
      |        P = Po * (V/Vo)^np * (1+Tp1.s)/(1+Tp2.s)
      |        Q = Qo * (V/Vo)^nq * (1+Tq1.s)/(1+Tq2.s)
      |   if V<Vmin
      |      Same equations with np=nq=2 (constant impedance load)
      mask init: same as ng_pv_dynamic_dbus_p_1_sm_ng/SM_NG/Single-Phase Dynamic Load32
      mask Help: helpview(psbhelp)
      mask Callback ExternalControl: powericon('ThreePhaseDynamicLoadCback',gcb);
      mask Display:
      | plot(.2*[0 3.5 5 2 0], .2*[1 1 4.5 4.5 1])
      | plot(.2*[1.7 3.5], .2*[1 4.5])
      | plot(.2*[1.1 4.3], .2*[3 3])
      | plot(.2*[.6 3.9], .2*[2 2])
      | plot(.2*[1.7 4.7], .2*[3.9 3.9])
  Single-Phase Dynamic Load35 : Subsystem  DialogController=POWERSYS.PowerSysDialog  mask(Single-Phase Dynamic Load){NominalVoltage=|, ActiveReactivePowers=|, PositiveSequence=[1 0], ExternalControl=on, NpNq=[np nq], TimeConstants=[0  0  0  0], MinimumVoltage=Vmin, LoadFlowParameters=[4,0,0,0,0]}
      mask NominalVoltage=|
      | [7967.43
      | 60 ]
      mask ActiveReactivePowers=|
      | [-22406.000
      | 7310.955]
      mask prompts: NominalVoltage "Nominal voltage and frequency  [Vn(Vrms) fn(Hz)]:"; ActiveReactivePowers "Active and reactive power at initial voltage [Po(W) Qo(var)]:"; PositiveSequence "Initial voltage Vo [Mag(pu) Phase (deg.)]:"; ExternalControl "External control of PQ"; NpNq "Parameters [ np  nq ]:"; TimeConstants "Time constants [Tp1 Tp2 Tq1 Tq2]  (s):"; MinimumVoltage "Minimum voltage Vmin (pu):"; LoadFlowParameters "Load Flow parameters"
      mask help:
      | Implements a single-phase dynamic load. Active  power P and reactive
      | power Q absorbed by the load vary as function of voltage V  according to the
      | following equations:
      |
      |   If V>Vmin, P and Q vary as follows:
      |        P = Po * (V/Vo)^np * (1+Tp1.s)/(1+Tp2.s)
      |        Q = Qo * (V/Vo)^nq * (1+Tq1.s)/(1+Tq2.s)
      |   if V<Vmin
      |      Same equations with np=nq=2 (constant impedance load)
      mask init: same as ng_pv_dynamic_dbus_p_1_sm_ng/SM_NG/Single-Phase Dynamic Load32
      mask Help: helpview(psbhelp)
      mask Callback ExternalControl: powericon('ThreePhaseDynamicLoadCback',gcb);
      mask Display:
      | plot(.2*[0 3.5 5 2 0], .2*[1 1 4.5 4.5 1])
      | plot(.2*[1.7 3.5], .2*[1 4.5])
      | plot(.2*[1.1 4.3], .2*[3 3])
      | plot(.2*[.6 3.9], .2*[2 2])
      | plot(.2*[1.7 4.7], .2*[3.9 3.9])
  Single-Phase Dynamic Load36 : Subsystem  DialogController=POWERSYS.PowerSysDialog  mask(Single-Phase Dynamic Load){NominalVoltage=[7967.43 60 ], ActiveReactivePowers=|, PositiveSequence=[1 0], ExternalControl=on, NpNq=[np nq], TimeConstants=[0  0  0  0], MinimumVoltage=Vmin, LoadFlowParameters=[4,0,0,0,0]}
      mask ActiveReactivePowers=|
      | [-67722.700
      | -9601.870]
      mask prompts: NominalVoltage "Nominal voltage and frequency  [Vn(Vrms) fn(Hz)]:"; ActiveReactivePowers "Active and reactive power at initial voltage [Po(W) Qo(var)]:"; PositiveSequence "Initial voltage Vo [Mag(pu) Phase (deg.)]:"; ExternalControl "External control of PQ"; NpNq "Parameters [ np  nq ]:"; TimeConstants "Time constants [Tp1 Tp2 Tq1 Tq2]  (s):"; MinimumVoltage "Minimum voltage Vmin (pu):"; LoadFlowParameters "Load Flow parameters"
      mask help:
      | Implements a single-phase dynamic load. Active  power P and reactive
      | power Q absorbed by the load vary as function of voltage V  according to the
      | following equations:
      |
      |   If V>Vmin, P and Q vary as follows:
      |        P = Po * (V/Vo)^np * (1+Tp1.s)/(1+Tp2.s)
      |        Q = Qo * (V/Vo)^nq * (1+Tq1.s)/(1+Tq2.s)
      |   if V<Vmin
      |      Same equations with np=nq=2 (constant impedance load)
      mask init: same as ng_pv_dynamic_dbus_p_1_sm_ng/SM_NG/Single-Phase Dynamic Load32
      mask Help: helpview(psbhelp)
      mask Callback ExternalControl: powericon('ThreePhaseDynamicLoadCback',gcb);
      mask Display:
      | plot(.2*[0 3.5 5 2 0], .2*[1 1 4.5 4.5 1])
      | plot(.2*[1.7 3.5], .2*[1 4.5])
      | plot(.2*[1.1 4.3], .2*[3 3])
      | plot(.2*[.6 3.9], .2*[2 2])
      | plot(.2*[1.7 4.7], .2*[3.9 3.9])
  Single-Phase Dynamic Load37 : Subsystem  DialogController=POWERSYS.PowerSysDialog  mask(Single-Phase Dynamic Load){NominalVoltage=|, ActiveReactivePowers=[-57616.400 -8183.737], PositiveSequence=[1 0], ExternalControl=on, NpNq=[np nq], TimeConstants=[0  0  0  0], MinimumVoltage=Vmin, LoadFlowParameters=[4,0,0,0,0]}
      mask NominalVoltage=|
      | [7967.43
      |  60 ]
      mask prompts: NominalVoltage "Nominal voltage and frequency  [Vn(Vrms) fn(Hz)]:"; ActiveReactivePowers "Active and reactive power at initial voltage [Po(W) Qo(var)]:"; PositiveSequence "Initial voltage Vo [Mag(pu) Phase (deg.)]:"; ExternalControl "External control of PQ"; NpNq "Parameters [ np  nq ]:"; TimeConstants "Time constants [Tp1 Tp2 Tq1 Tq2]  (s):"; MinimumVoltage "Minimum voltage Vmin (pu):"; LoadFlowParameters "Load Flow parameters"
      mask help:
      | Implements a single-phase dynamic load. Active  power P and reactive
      | power Q absorbed by the load vary as function of voltage V  according to the
      | following equations:
      |
      |   If V>Vmin, P and Q vary as follows:
      |        P = Po * (V/Vo)^np * (1+Tp1.s)/(1+Tp2.s)
      |        Q = Qo * (V/Vo)^nq * (1+Tq1.s)/(1+Tq2.s)
      |   if V<Vmin
      |      Same equations with np=nq=2 (constant impedance load)
      mask init: same as ng_pv_dynamic_dbus_p_1_sm_ng/SM_NG/Single-Phase Dynamic Load32
      mask Help: helpview(psbhelp)
      mask Callback ExternalControl: powericon('ThreePhaseDynamicLoadCback',gcb);
      mask Display:
      | plot(.2*[0 3.5 5 2 0], .2*[1 1 4.5 4.5 1])
      | plot(.2*[1.7 3.5], .2*[1 4.5])
      | plot(.2*[1.1 4.3], .2*[3 3])
      | plot(.2*[.6 3.9], .2*[2 2])
      | plot(.2*[1.7 4.7], .2*[3.9 3.9])
  Single-Phase Dynamic Load38 : Subsystem  DialogController=POWERSYS.PowerSysDialog  mask(Single-Phase Dynamic Load){NominalVoltage=|, ActiveReactivePowers=[-13034.700 1861.143], PositiveSequence=[1 0], ExternalControl=on, NpNq=[np nq], TimeConstants=[0  0  0  0], MinimumVoltage=Vmin, LoadFlowParameters=[4,0,0,0,0]}
      mask NominalVoltage=|
      | [7967.43
      |  60 ]
      mask prompts: NominalVoltage "Nominal voltage and frequency  [Vn(Vrms) fn(Hz)]:"; ActiveReactivePowers "Active and reactive power at initial voltage [Po(W) Qo(var)]:"; PositiveSequence "Initial voltage Vo [Mag(pu) Phase (deg.)]:"; ExternalControl "External control of PQ"; NpNq "Parameters [ np  nq ]:"; TimeConstants "Time constants [Tp1 Tp2 Tq1 Tq2]  (s):"; MinimumVoltage "Minimum voltage Vmin (pu):"; LoadFlowParameters "Load Flow parameters"
      mask help:
      | Implements a single-phase dynamic load. Active  power P and reactive
      | power Q absorbed by the load vary as function of voltage V  according to the
      | following equations:
      |
      |   If V>Vmin, P and Q vary as follows:
      |        P = Po * (V/Vo)^np * (1+Tp1.s)/(1+Tp2.s)
      |        Q = Qo * (V/Vo)^nq * (1+Tq1.s)/(1+Tq2.s)
      |   if V<Vmin
      |      Same equations with np=nq=2 (constant impedance load)
      mask init: same as ng_pv_dynamic_dbus_p_1_sm_ng/SM_NG/Single-Phase Dynamic Load32
      mask Help: helpview(psbhelp)
      mask Callback ExternalControl: powericon('ThreePhaseDynamicLoadCback',gcb);
      mask Display:
      | plot(.2*[0 3.5 5 2 0], .2*[1 1 4.5 4.5 1])
      | plot(.2*[1.7 3.5], .2*[1 4.5])
      | plot(.2*[1.1 4.3], .2*[3 3])
      | plot(.2*[.6 3.9], .2*[2 2])
      | plot(.2*[1.7 4.7], .2*[3.9 3.9])
  Single-Phase Dynamic Load39 : Subsystem  DialogController=POWERSYS.PowerSysDialog  mask(Single-Phase Dynamic Load){NominalVoltage=|, ActiveReactivePowers=|, PositiveSequence=[1 0], ExternalControl=on, NpNq=[np nq], TimeConstants=[0  0  0  0], MinimumVoltage=Vmin, LoadFlowParameters=[4,0,0,0,0]}
      mask NominalVoltage=|
      | [7967.43
      |  60 ]
      mask ActiveReactivePowers=|
      | [-51807.900
      | -7365.107]
      mask prompts: NominalVoltage "Nominal voltage and frequency  [Vn(Vrms) fn(Hz)]:"; ActiveReactivePowers "Active and reactive power at initial voltage [Po(W) Qo(var)]:"; PositiveSequence "Initial voltage Vo [Mag(pu) Phase (deg.)]:"; ExternalControl "External control of PQ"; NpNq "Parameters [ np  nq ]:"; TimeConstants "Time constants [Tp1 Tp2 Tq1 Tq2]  (s):"; MinimumVoltage "Minimum voltage Vmin (pu):"; LoadFlowParameters "Load Flow parameters"
      mask help:
      | Implements a single-phase dynamic load. Active  power P and reactive
      | power Q absorbed by the load vary as function of voltage V  according to the
      | following equations:
      |
      |   If V>Vmin, P and Q vary as follows:
      |        P = Po * (V/Vo)^np * (1+Tp1.s)/(1+Tp2.s)
      |        Q = Qo * (V/Vo)^nq * (1+Tq1.s)/(1+Tq2.s)
      |   if V<Vmin
      |      Same equations with np=nq=2 (constant impedance load)
      mask init: same as ng_pv_dynamic_dbus_p_1_sm_ng/SM_NG/Single-Phase Dynamic Load32
      mask Help: helpview(psbhelp)
      mask Callback ExternalControl: powericon('ThreePhaseDynamicLoadCback',gcb);
      mask Display:
      | plot(.2*[0 3.5 5 2 0], .2*[1 1 4.5 4.5 1])
      | plot(.2*[1.7 3.5], .2*[1 4.5])
      | plot(.2*[1.1 4.3], .2*[3 3])
      | plot(.2*[.6 3.9], .2*[2 2])
      | plot(.2*[1.7 4.7], .2*[3.9 3.9])
  Single-Phase Dynamic Load40 : Subsystem  DialogController=POWERSYS.PowerSysDialog  mask(Single-Phase Dynamic Load){NominalVoltage=|, ActiveReactivePowers=|, PositiveSequence=[1 0], ExternalControl=on, NpNq=[np nq], TimeConstants=[0  0  0  0], MinimumVoltage=Vmin, LoadFlowParameters=[4,0,0,0,0]}
      mask NominalVoltage=|
      | [7967.43
      |  60 ]
      mask ActiveReactivePowers=|
      | [-18221.200
      | -2652.826]
      mask prompts: NominalVoltage "Nominal voltage and frequency  [Vn(Vrms) fn(Hz)]:"; ActiveReactivePowers "Active and reactive power at initial voltage [Po(W) Qo(var)]:"; PositiveSequence "Initial voltage Vo [Mag(pu) Phase (deg.)]:"; ExternalControl "External control of PQ"; NpNq "Parameters [ np  nq ]:"; TimeConstants "Time constants [Tp1 Tp2 Tq1 Tq2]  (s):"; MinimumVoltage "Minimum voltage Vmin (pu):"; LoadFlowParameters "Load Flow parameters"
      mask help:
      | Implements a single-phase dynamic load. Active  power P and reactive
      | power Q absorbed by the load vary as function of voltage V  according to the
      | following equations:
      |
      |   If V>Vmin, P and Q vary as follows:
      |        P = Po * (V/Vo)^np * (1+Tp1.s)/(1+Tp2.s)
      |        Q = Qo * (V/Vo)^nq * (1+Tq1.s)/(1+Tq2.s)
      |   if V<Vmin
      |      Same equations with np=nq=2 (constant impedance load)
      mask init: same as ng_pv_dynamic_dbus_p_1_sm_ng/SM_NG/Single-Phase Dynamic Load32
      mask Help: helpview(psbhelp)
      mask Callback ExternalControl: powericon('ThreePhaseDynamicLoadCback',gcb);
      mask Display:
      | plot(.2*[0 3.5 5 2 0], .2*[1 1 4.5 4.5 1])
      | plot(.2*[1.7 3.5], .2*[1 4.5])
      | plot(.2*[1.1 4.3], .2*[3 3])
      | plot(.2*[.6 3.9], .2*[2 2])
      | plot(.2*[1.7 4.7], .2*[3.9 3.9])
  Single-Phase Dynamic Load41 : Subsystem  DialogController=POWERSYS.PowerSysDialog  mask(Single-Phase Dynamic Load){NominalVoltage=|, ActiveReactivePowers=[-119379.000 21541.648], PositiveSequence=[1 0], ExternalControl=on, NpNq=[np nq], TimeConstants=[0  0  0  0], MinimumVoltage=Vmin, LoadFlowParameters=[4,0,0,0,0]}
      mask NominalVoltage=|
      | [7967.43
      |  60 ]
      mask prompts: NominalVoltage "Nominal voltage and frequency  [Vn(Vrms) fn(Hz)]:"; ActiveReactivePowers "Active and reactive power at initial voltage [Po(W) Qo(var)]:"; PositiveSequence "Initial voltage Vo [Mag(pu) Phase (deg.)]:"; ExternalControl "External control of PQ"; NpNq "Parameters [ np  nq ]:"; TimeConstants "Time constants [Tp1 Tp2 Tq1 Tq2]  (s):"; MinimumVoltage "Minimum voltage Vmin (pu):"; LoadFlowParameters "Load Flow parameters"
      mask help:
      | Implements a single-phase dynamic load. Active  power P and reactive
      | power Q absorbed by the load vary as function of voltage V  according to the
      | following equations:
      |
      |   If V>Vmin, P and Q vary as follows:
      |        P = Po * (V/Vo)^np * (1+Tp1.s)/(1+Tp2.s)
      |        Q = Qo * (V/Vo)^nq * (1+Tq1.s)/(1+Tq2.s)
      |   if V<Vmin
      |      Same equations with np=nq=2 (constant impedance load)
      mask init: same as ng_pv_dynamic_dbus_p_1_sm_ng/SM_NG/Single-Phase Dynamic Load32
      mask Help: helpview(psbhelp)
      mask Callback ExternalControl: powericon('ThreePhaseDynamicLoadCback',gcb);
      mask Display:
      | plot(.2*[0 3.5 5 2 0], .2*[1 1 4.5 4.5 1])
      | plot(.2*[1.7 3.5], .2*[1 4.5])
      | plot(.2*[1.1 4.3], .2*[3 3])
      | plot(.2*[.6 3.9], .2*[2 2])
      | plot(.2*[1.7 4.7], .2*[3.9 3.9])
  Single-Phase Dynamic Load42 : Subsystem  DialogController=POWERSYS.PowerSysDialog  mask(Single-Phase Dynamic Load){NominalVoltage=[7967.43 60 ], ActiveReactivePowers=[-29638.700  -4207.799], PositiveSequence=[1 0], ExternalControl=on, NpNq=[np nq], TimeConstants=[0  0  0  0], MinimumVoltage=Vmin, LoadFlowParameters=[4,0,0,0,0]}
      mask prompts: NominalVoltage "Nominal voltage and frequency  [Vn(Vrms) fn(Hz)]:"; ActiveReactivePowers "Active and reactive power at initial voltage [Po(W) Qo(var)]:"; PositiveSequence "Initial voltage Vo [Mag(pu) Phase (deg.)]:"; ExternalControl "External control of PQ"; NpNq "Parameters [ np  nq ]:"; TimeConstants "Time constants [Tp1 Tp2 Tq1 Tq2]  (s):"; MinimumVoltage "Minimum voltage Vmin (pu):"; LoadFlowParameters "Load Flow parameters"
      mask help:
      | Implements a single-phase dynamic load. Active  power P and reactive
      | power Q absorbed by the load vary as function of voltage V  according to the
      | following equations:
      |
      |   If V>Vmin, P and Q vary as follows:
      |        P = Po * (V/Vo)^np * (1+Tp1.s)/(1+Tp2.s)
      |        Q = Qo * (V/Vo)^nq * (1+Tq1.s)/(1+Tq2.s)
      |   if V<Vmin
      |      Same equations with np=nq=2 (constant impedance load)
      mask init: same as ng_pv_dynamic_dbus_p_1_sm_ng/SM_NG/Single-Phase Dynamic Load32
      mask Help: helpview(psbhelp)
      mask Callback ExternalControl: powericon('ThreePhaseDynamicLoadCback',gcb);
      mask Display:
      | plot(.2*[0 3.5 5 2 0], .2*[1 1 4.5 4.5 1])
      | 
      | plot(.2*[1.7 3.5], .2*[1 4.5])
      | 
      | plot(.2*[1.1 4.3], .2*[3 3])
      | 
      | plot(.2*[.6 3.9], .2*[2 2])
      | 
      | plot(.2*[1.7 4.7], .2*[3.9 3.9])
  Single-Phase Dynamic Load43 : Subsystem  DialogController=POWERSYS.PowerSysDialog  mask(Single-Phase Dynamic Load){NominalVoltage=|, ActiveReactivePowers=[-53874.300 10730.813], PositiveSequence=[1 0], ExternalControl=on, NpNq=[np nq], TimeConstants=[0  0  0  0], MinimumVoltage=Vmin, LoadFlowParameters=[4,0,0,0,0]}
      mask NominalVoltage=|
      | [7967.43
      |  60 ]
      mask prompts: NominalVoltage "Nominal voltage and frequency  [Vn(Vrms) fn(Hz)]:"; ActiveReactivePowers "Active and reactive power at initial voltage [Po(W) Qo(var)]:"; PositiveSequence "Initial voltage Vo [Mag(pu) Phase (deg.)]:"; ExternalControl "External control of PQ"; NpNq "Parameters [ np  nq ]:"; TimeConstants "Time constants [Tp1 Tp2 Tq1 Tq2]  (s):"; MinimumVoltage "Minimum voltage Vmin (pu):"; LoadFlowParameters "Load Flow parameters"
      mask help:
      | Implements a single-phase dynamic load. Active  power P and reactive
      | power Q absorbed by the load vary as function of voltage V  according to the
      | following equations:
      |
      |   If V>Vmin, P and Q vary as follows:
      |        P = Po * (V/Vo)^np * (1+Tp1.s)/(1+Tp2.s)
      |        Q = Qo * (V/Vo)^nq * (1+Tq1.s)/(1+Tq2.s)
      |   if V<Vmin
      |      Same equations with np=nq=2 (constant impedance load)
      mask init: same as ng_pv_dynamic_dbus_p_1_sm_ng/SM_NG/Single-Phase Dynamic Load32
      mask Help: helpview(psbhelp)
      mask Callback ExternalControl: powericon('ThreePhaseDynamicLoadCback',gcb);
      mask Display:
      | plot(.2*[0 3.5 5 2 0], .2*[1 1 4.5 4.5 1])
      | plot(.2*[1.7 3.5], .2*[1 4.5])
      | plot(.2*[1.1 4.3], .2*[3 3])
      | plot(.2*[.6 3.9], .2*[2 2])
      | plot(.2*[1.7 4.7], .2*[3.9 3.9])
  Single-Phase Dynamic Load44 : Subsystem  DialogController=POWERSYS.PowerSysDialog  mask(Single-Phase Dynamic Load){NominalVoltage=|, ActiveReactivePowers=[-44033.300 -6802.859], PositiveSequence=[1 0], ExternalControl=on, NpNq=[np nq], TimeConstants=[0  0  0  0], MinimumVoltage=Vmin, LoadFlowParameters=[4,0,0,0,0]}
      mask NominalVoltage=|
      | [7967.00
      |  60 ]
      mask prompts: NominalVoltage "Nominal voltage and frequency  [Vn(Vrms) fn(Hz)]:"; ActiveReactivePowers "Active and reactive power at initial voltage [Po(W) Qo(var)]:"; PositiveSequence "Initial voltage Vo [Mag(pu) Phase (deg.)]:"; ExternalControl "External control of PQ"; NpNq "Parameters [ np  nq ]:"; TimeConstants "Time constants [Tp1 Tp2 Tq1 Tq2]  (s):"; MinimumVoltage "Minimum voltage Vmin (pu):"; LoadFlowParameters "Load Flow parameters"
      mask help:
      | Implements a single-phase dynamic load. Active  power P and reactive
      | power Q absorbed by the load vary as function of voltage V  according to the
      | following equations:
      |
      |   If V>Vmin, P and Q vary as follows:
      |        P = Po * (V/Vo)^np * (1+Tp1.s)/(1+Tp2.s)
      |        Q = Qo * (V/Vo)^nq * (1+Tq1.s)/(1+Tq2.s)
      |   if V<Vmin
      |      Same equations with np=nq=2 (constant impedance load)
      mask init: same as ng_pv_dynamic_dbus_p_1_sm_ng/SM_NG/Single-Phase Dynamic Load32
      mask Help: helpview(psbhelp)
      mask Callback ExternalControl: powericon('ThreePhaseDynamicLoadCback',gcb);
      mask Display:
      | plot(.2*[0 3.5 5 2 0], .2*[1 1 4.5 4.5 1])
      | plot(.2*[1.7 3.5], .2*[1 4.5])
      | plot(.2*[1.1 4.3], .2*[3 3])
      | plot(.2*[.6 3.9], .2*[2 2])
      | plot(.2*[1.7 4.7], .2*[3.9 3.9])
  Single-Phase Dynamic Load45 : Subsystem  DialogController=POWERSYS.PowerSysDialog  mask(Single-Phase Dynamic Load){NominalVoltage=|, ActiveReactivePowers=|, PositiveSequence=[1 0], ExternalControl=on, NpNq=[np nq], TimeConstants=[0  0  0  0], MinimumVoltage=Vmin, LoadFlowParameters=[4,0,0,0,0]}
      mask NominalVoltage=|
      | [7967.00
      |  60 ]
      mask ActiveReactivePowers=|
      | [-150415.000
      | -24442.388]
      mask prompts: NominalVoltage "Nominal voltage and frequency  [Vn(Vrms) fn(Hz)]:"; ActiveReactivePowers "Active and reactive power at initial voltage [Po(W) Qo(var)]:"; PositiveSequence "Initial voltage Vo [Mag(pu) Phase (deg.)]:"; ExternalControl "External control of PQ"; NpNq "Parameters [ np  nq ]:"; TimeConstants "Time constants [Tp1 Tp2 Tq1 Tq2]  (s):"; MinimumVoltage "Minimum voltage Vmin (pu):"; LoadFlowParameters "Load Flow parameters"
      mask help:
      | Implements a single-phase dynamic load. Active  power P and reactive
      | power Q absorbed by the load vary as function of voltage V  according to the
      | following equations:
      |
      |   If V>Vmin, P and Q vary as follows:
      |        P = Po * (V/Vo)^np * (1+Tp1.s)/(1+Tp2.s)
      |        Q = Qo * (V/Vo)^nq * (1+Tq1.s)/(1+Tq2.s)
      |   if V<Vmin
      |      Same equations with np=nq=2 (constant impedance load)
      mask init: same as ng_pv_dynamic_dbus_p_1_sm_ng/SM_NG/Single-Phase Dynamic Load32
      mask Help: helpview(psbhelp)
      mask Callback ExternalControl: powericon('ThreePhaseDynamicLoadCback',gcb);
      mask Display:
      | plot(.2*[0 3.5 5 2 0], .2*[1 1 4.5 4.5 1])
      | plot(.2*[1.7 3.5], .2*[1 4.5])
      | plot(.2*[1.1 4.3], .2*[3 3])
      | plot(.2*[.6 3.9], .2*[2 2])
      | plot(.2*[1.7 4.7], .2*[3.9 3.9])
  Single-Phase Dynamic Load46 : Subsystem  DialogController=POWERSYS.PowerSysDialog  mask(Single-Phase Dynamic Load){NominalVoltage=|, ActiveReactivePowers=|, PositiveSequence=[1 0], ExternalControl=on, NpNq=[np nq], TimeConstants=[0  0  0  0], MinimumVoltage=Vmin, LoadFlowParameters=[4,0,0,0,0]}
      mask NominalVoltage=|
      | [7967.00
      |  60 ]
      mask ActiveReactivePowers=|
      | [-21237.500
      | -6400.072]
      mask prompts: NominalVoltage "Nominal voltage and frequency  [Vn(Vrms) fn(Hz)]:"; ActiveReactivePowers "Active and reactive power at initial voltage [Po(W) Qo(var)]:"; PositiveSequence "Initial voltage Vo [Mag(pu) Phase (deg.)]:"; ExternalControl "External control of PQ"; NpNq "Parameters [ np  nq ]:"; TimeConstants "Time constants [Tp1 Tp2 Tq1 Tq2]  (s):"; MinimumVoltage "Minimum voltage Vmin (pu):"; LoadFlowParameters "Load Flow parameters"
      mask help:
      | Implements a single-phase dynamic load. Active  power P and reactive
      | power Q absorbed by the load vary as function of voltage V  according to the
      | following equations:
      |
      |   If V>Vmin, P and Q vary as follows:
      |        P = Po * (V/Vo)^np * (1+Tp1.s)/(1+Tp2.s)
      |        Q = Qo * (V/Vo)^nq * (1+Tq1.s)/(1+Tq2.s)
      |   if V<Vmin
      |      Same equations with np=nq=2 (constant impedance load)
      mask init: same as ng_pv_dynamic_dbus_p_1_sm_ng/SM_NG/Single-Phase Dynamic Load32
      mask Help: helpview(psbhelp)
      mask Callback ExternalControl: powericon('ThreePhaseDynamicLoadCback',gcb);
      mask Display:
      | plot(.2*[0 3.5 5 2 0], .2*[1 1 4.5 4.5 1])
      | plot(.2*[1.7 3.5], .2*[1 4.5])
      | plot(.2*[1.1 4.3], .2*[3 3])
      | plot(.2*[.6 3.9], .2*[2 2])
      | plot(.2*[1.7 4.7], .2*[3.9 3.9])
  Single-Phase Dynamic Load47 : Subsystem  DialogController=POWERSYS.PowerSysDialog  mask(Single-Phase Dynamic Load){NominalVoltage=|, ActiveReactivePowers=[-34508.300 4892.517], PositiveSequence=[1 0], ExternalControl=on, NpNq=[np nq], TimeConstants=[0  0  0  0], MinimumVoltage=Vmin, LoadFlowParameters=[4,0,0,0,0]}
      mask NominalVoltage=|
      | [7967.43
      |  60 ]
      mask prompts: NominalVoltage "Nominal voltage and frequency  [Vn(Vrms) fn(Hz)]:"; ActiveReactivePowers "Active and reactive power at initial voltage [Po(W) Qo(var)]:"; PositiveSequence "Initial voltage Vo [Mag(pu) Phase (deg.)]:"; ExternalControl "External control of PQ"; NpNq "Parameters [ np  nq ]:"; TimeConstants "Time constants [Tp1 Tp2 Tq1 Tq2]  (s):"; MinimumVoltage "Minimum voltage Vmin (pu):"; LoadFlowParameters "Load Flow parameters"
      mask help:
      | Implements a single-phase dynamic load. Active  power P and reactive
      | power Q absorbed by the load vary as function of voltage V  according to the
      | following equations:
      |
      |   If V>Vmin, P and Q vary as follows:
      |        P = Po * (V/Vo)^np * (1+Tp1.s)/(1+Tp2.s)
      |        Q = Qo * (V/Vo)^nq * (1+Tq1.s)/(1+Tq2.s)
      |   if V<Vmin
      |      Same equations with np=nq=2 (constant impedance load)
      mask init: same as ng_pv_dynamic_dbus_p_1_sm_ng/SM_NG/Single-Phase Dynamic Load32
      mask Help: helpview(psbhelp)
      mask Callback ExternalControl: powericon('ThreePhaseDynamicLoadCback',gcb);
      mask Display:
      | plot(.2*[0 3.5 5 2 0], .2*[1 1 4.5 4.5 1])
      | plot(.2*[1.7 3.5], .2*[1 4.5])
      | plot(.2*[1.1 4.3], .2*[3 3])
      | plot(.2*[.6 3.9], .2*[2 2])
      | plot(.2*[1.7 4.7], .2*[3.9 3.9])
  Single-Phase Dynamic Load48 : Subsystem  DialogController=POWERSYS.PowerSysDialog  mask(Single-Phase Dynamic Load){NominalVoltage=[ 7967.43 60 ], ActiveReactivePowers=|, PositiveSequence=[1 0], ExternalControl=on, NpNq=[np nq], TimeConstants=[0  0  0  0], MinimumVoltage=Vmin, LoadFlowParameters=[4,0,0,0,0]}
      mask ActiveReactivePowers=|
      | [-22450.700
      | 3182.886]
      mask prompts: NominalVoltage "Nominal voltage and frequency  [Vn(Vrms) fn(Hz)]:"; ActiveReactivePowers "Active and reactive power at initial voltage [Po(W) Qo(var)]:"; PositiveSequence "Initial voltage Vo [Mag(pu) Phase (deg.)]:"; ExternalControl "External control of PQ"; NpNq "Parameters [ np  nq ]:"; TimeConstants "Time constants [Tp1 Tp2 Tq1 Tq2]  (s):"; MinimumVoltage "Minimum voltage Vmin (pu):"; LoadFlowParameters "Load Flow parameters"
      mask help:
      | Implements a single-phase dynamic load. Active  power P and reactive
      | power Q absorbed by the load vary as function of voltage V  according to the
      | following equations:
      |
      |   If V>Vmin, P and Q vary as follows:
      |        P = Po * (V/Vo)^np * (1+Tp1.s)/(1+Tp2.s)
      |        Q = Qo * (V/Vo)^nq * (1+Tq1.s)/(1+Tq2.s)
      |   if V<Vmin
      |      Same equations with np=nq=2 (constant impedance load)
      mask init: same as ng_pv_dynamic_dbus_p_1_sm_ng/SM_NG/Single-Phase Dynamic Load32
      mask Help: helpview(psbhelp)
      mask Callback ExternalControl: powericon('ThreePhaseDynamicLoadCback',gcb);
      mask Display:
      | plot(.2*[0 3.5 5 2 0], .2*[1 1 4.5 4.5 1])
      | plot(.2*[1.7 3.5], .2*[1 4.5])
      | plot(.2*[1.1 4.3], .2*[3 3])
      | plot(.2*[.6 3.9], .2*[2 2])
      | plot(.2*[1.7 4.7], .2*[3.9 3.9])
  Single-Phase Dynamic Load49 : Subsystem  DialogController=POWERSYS.PowerSysDialog  mask(Single-Phase Dynamic Load){NominalVoltage=|, ActiveReactivePowers=|, PositiveSequence=[1 0], ExternalControl=on, NpNq=[np nq], TimeConstants=[0  0  0  0], MinimumVoltage=Vmin, LoadFlowParameters=[4,0,0,0,0]}
      mask NominalVoltage=|
      | [ 7967.43
      |  60 ]
      mask ActiveReactivePowers=|
      | [-9065.390
      | 1285.213]
      mask prompts: NominalVoltage "Nominal voltage and frequency  [Vn(Vrms) fn(Hz)]:"; ActiveReactivePowers "Active and reactive power at initial voltage [Po(W) Qo(var)]:"; PositiveSequence "Initial voltage Vo [Mag(pu) Phase (deg.)]:"; ExternalControl "External control of PQ"; NpNq "Parameters [ np  nq ]:"; TimeConstants "Time constants [Tp1 Tp2 Tq1 Tq2]  (s):"; MinimumVoltage "Minimum voltage Vmin (pu):"; LoadFlowParameters "Load Flow parameters"
      mask help:
      | Implements a single-phase dynamic load. Active  power P and reactive
      | power Q absorbed by the load vary as function of voltage V  according to the
      | following equations:
      |
      |   If V>Vmin, P and Q vary as follows:
      |        P = Po * (V/Vo)^np * (1+Tp1.s)/(1+Tp2.s)
      |        Q = Qo * (V/Vo)^nq * (1+Tq1.s)/(1+Tq2.s)
      |   if V<Vmin
      |      Same equations with np=nq=2 (constant impedance load)
      mask init: same as ng_pv_dynamic_dbus_p_1_sm_ng/SM_NG/Single-Phase Dynamic Load32
      mask Help: helpview(psbhelp)
      mask Callback ExternalControl: powericon('ThreePhaseDynamicLoadCback',gcb);
      mask Display:
      | plot(.2*[0 3.5 5 2 0], .2*[1 1 4.5 4.5 1])
      | plot(.2*[1.7 3.5], .2*[1 4.5])
      | plot(.2*[1.1 4.3], .2*[3 3])
      | plot(.2*[.6 3.9], .2*[2 2])
      | plot(.2*[1.7 4.7], .2*[3.9 3.9])
  Single-Phase Dynamic Load50 : Subsystem  DialogController=POWERSYS.PowerSysDialog  mask(Single-Phase Dynamic Load){NominalVoltage=[7967.43 60 ], ActiveReactivePowers=[-1001990.000 143475.169], PositiveSequence=[1 0], ExternalControl=on, NpNq=[np nq], TimeConstants=[0  0  0  0], MinimumVoltage=Vmin, LoadFlowParameters=[4,0,0,0,0]}
      mask prompts: NominalVoltage "Nominal voltage and frequency  [Vn(Vrms) fn(Hz)]:"; ActiveReactivePowers "Active and reactive power at initial voltage [Po(W) Qo(var)]:"; PositiveSequence "Initial voltage Vo [Mag(pu) Phase (deg.)]:"; ExternalControl "External control of PQ"; NpNq "Parameters [ np  nq ]:"; TimeConstants "Time constants [Tp1 Tp2 Tq1 Tq2]  (s):"; MinimumVoltage "Minimum voltage Vmin (pu):"; LoadFlowParameters "Load Flow parameters"
      mask help:
      | Implements a single-phase dynamic load. Active  power P and reactive
      | power Q absorbed by the load vary as function of voltage V  according to the
      | following equations:
      |
      |   If V>Vmin, P and Q vary as follows:
      |        P = Po * (V/Vo)^np * (1+Tp1.s)/(1+Tp2.s)
      |        Q = Qo * (V/Vo)^nq * (1+Tq1.s)/(1+Tq2.s)
      |   if V<Vmin
      |      Same equations with np=nq=2 (constant impedance load)
      mask init: same as ng_pv_dynamic_dbus_p_1_sm_ng/SM_NG/Single-Phase Dynamic Load32
      mask Help: helpview(psbhelp)
      mask Callback ExternalControl: powericon('ThreePhaseDynamicLoadCback',gcb);
      mask Display:
      | plot(.2*[0 3.5 5 2 0], .2*[1 1 4.5 4.5 1])
      | plot(.2*[1.7 3.5], .2*[1 4.5])
      | plot(.2*[1.1 4.3], .2*[3 3])
      | plot(.2*[.6 3.9], .2*[2 2])
      | plot(.2*[1.7 4.7], .2*[3.9 3.9])
  Single-Phase Dynamic Load51 : Subsystem  DialogController=POWERSYS.PowerSysDialog  mask(Single-Phase Dynamic Load){NominalVoltage=[7967.43 60 ], ActiveReactivePowers=|, PositiveSequence=[1 0], ExternalControl=on, NpNq=[np nq], TimeConstants=[0  0  0  0], MinimumVoltage=Vmin, LoadFlowParameters=[4,0,0,0,0]}
      mask ActiveReactivePowers=|
      | [-1018490.000
      | -144503.412]
      mask prompts: NominalVoltage "Nominal voltage and frequency  [Vn(Vrms) fn(Hz)]:"; ActiveReactivePowers "Active and reactive power at initial voltage [Po(W) Qo(var)]:"; PositiveSequence "Initial voltage Vo [Mag(pu) Phase (deg.)]:"; ExternalControl "External control of PQ"; NpNq "Parameters [ np  nq ]:"; TimeConstants "Time constants [Tp1 Tp2 Tq1 Tq2]  (s):"; MinimumVoltage "Minimum voltage Vmin (pu):"; LoadFlowParameters "Load Flow parameters"
      mask help:
      | Implements a single-phase dynamic load. Active  power P and reactive
      | power Q absorbed by the load vary as function of voltage V  according to the
      | following equations:
      |
      |   If V>Vmin, P and Q vary as follows:
      |        P = Po * (V/Vo)^np * (1+Tp1.s)/(1+Tp2.s)
      |        Q = Qo * (V/Vo)^nq * (1+Tq1.s)/(1+Tq2.s)
      |   if V<Vmin
      |      Same equations with np=nq=2 (constant impedance load)
      mask init: same as ng_pv_dynamic_dbus_p_1_sm_ng/SM_NG/Single-Phase Dynamic Load32
      mask Help: helpview(psbhelp)
      mask Callback ExternalControl: powericon('ThreePhaseDynamicLoadCback',gcb);
      mask Display:
      | plot(.2*[0 3.5 5 2 0], .2*[1 1 4.5 4.5 1])
      | plot(.2*[1.7 3.5], .2*[1 4.5])
      | plot(.2*[1.1 4.3], .2*[3 3])
      | plot(.2*[.6 3.9], .2*[2 2])
      | plot(.2*[1.7 4.7], .2*[3.9 3.9])
  Single-Phase Dynamic Load52 : Subsystem  DialogController=POWERSYS.PowerSysDialog  mask(Single-Phase Dynamic Load){NominalVoltage=[7967.43 60 ], ActiveReactivePowers=[-983676.000 139461.852], PositiveSequence=[1 0], ExternalControl=on, NpNq=[np nq], TimeConstants=[0  0  0  0], MinimumVoltage=Vmin, LoadFlowParameters=[4,0,0,0,0]}
      mask prompts: NominalVoltage "Nominal voltage and frequency  [Vn(Vrms) fn(Hz)]:"; ActiveReactivePowers "Active and reactive power at initial voltage [Po(W) Qo(var)]:"; PositiveSequence "Initial voltage Vo [Mag(pu) Phase (deg.)]:"; ExternalControl "External control of PQ"; NpNq "Parameters [ np  nq ]:"; TimeConstants "Time constants [Tp1 Tp2 Tq1 Tq2]  (s):"; MinimumVoltage "Minimum voltage Vmin (pu):"; LoadFlowParameters "Load Flow parameters"
      mask help:
      | Implements a single-phase dynamic load. Active  power P and reactive
      | power Q absorbed by the load vary as function of voltage V  according to the
      | following equations:
      |
      |   If V>Vmin, P and Q vary as follows:
      |        P = Po * (V/Vo)^np * (1+Tp1.s)/(1+Tp2.s)
      |        Q = Qo * (V/Vo)^nq * (1+Tq1.s)/(1+Tq2.s)
      |   if V<Vmin
      |      Same equations with np=nq=2 (constant impedance load)
      mask init: same as ng_pv_dynamic_dbus_p_1_sm_ng/SM_NG/Single-Phase Dynamic Load32
      mask Help: helpview(psbhelp)
      mask Callback ExternalControl: powericon('ThreePhaseDynamicLoadCback',gcb);
      mask Display:
      | plot(.2*[0 3.5 5 2 0], .2*[1 1 4.5 4.5 1])
      | plot(.2*[1.7 3.5], .2*[1 4.5])
      | plot(.2*[1.1 4.3], .2*[3 3])
      | plot(.2*[.6 3.9], .2*[2 2])
      | plot(.2*[1.7 4.7], .2*[3.9 3.9])
  Single-Phase Dynamic Load53 : Subsystem  DialogController=POWERSYS.PowerSysDialog  mask(Single-Phase Dynamic Load){NominalVoltage=[7967.43 60 ], ActiveReactivePowers=[-2219.570 -318.814], PositiveSequence=[1 0], ExternalControl=on, NpNq=[np nq], TimeConstants=[0  0  0  0], MinimumVoltage=Vmin, LoadFlowParameters=[4,0,0,0,0]}
      mask prompts: NominalVoltage "Nominal voltage and frequency  [Vn(Vrms) fn(Hz)]:"; ActiveReactivePowers "Active and reactive power at initial voltage [Po(W) Qo(var)]:"; PositiveSequence "Initial voltage Vo [Mag(pu) Phase (deg.)]:"; ExternalControl "External control of PQ"; NpNq "Parameters [ np  nq ]:"; TimeConstants "Time constants [Tp1 Tp2 Tq1 Tq2]  (s):"; MinimumVoltage "Minimum voltage Vmin (pu):"; LoadFlowParameters "Load Flow parameters"
      mask help:
      | Implements a single-phase dynamic load. Active  power P and reactive
      | power Q absorbed by the load vary as function of voltage V  according to the
      | following equations:
      |
      |   If V>Vmin, P and Q vary as follows:
      |        P = Po * (V/Vo)^np * (1+Tp1.s)/(1+Tp2.s)
      |        Q = Qo * (V/Vo)^nq * (1+Tq1.s)/(1+Tq2.s)
      |   if V<Vmin
      |      Same equations with np=nq=2 (constant impedance load)
      mask init: same as ng_pv_dynamic_dbus_p_1_sm_ng/SM_NG/Single-Phase Dynamic Load32
      mask Help: helpview(psbhelp)
      mask Callback ExternalControl: powericon('ThreePhaseDynamicLoadCback',gcb);
      mask Display:
      | plot(.2*[0 3.5 5 2 0], .2*[1 1 4.5 4.5 1])
      | plot(.2*[1.7 3.5], .2*[1 4.5])
      | plot(.2*[1.1 4.3], .2*[3 3])
      | plot(.2*[.6 3.9], .2*[2 2])
      | plot(.2*[1.7 4.7], .2*[3.9 3.9])
  Single-Phase Dynamic Load54 : Subsystem  DialogController=POWERSYS.PowerSysDialog  mask(Single-Phase Dynamic Load){NominalVoltage=|, ActiveReactivePowers=[-4738.140  2577.318], PositiveSequence=[1 0], ExternalControl=on, NpNq=[np nq], TimeConstants=[0  0  0  0], MinimumVoltage=Vmin, LoadFlowParameters=[4,0,0,0,0]}
      mask NominalVoltage=|
      | [7967.43
      | 60 ]
      mask prompts: NominalVoltage "Nominal voltage and frequency  [Vn(Vrms) fn(Hz)]:"; ActiveReactivePowers "Active and reactive power at initial voltage [Po(W) Qo(var)]:"; PositiveSequence "Initial voltage Vo [Mag(pu) Phase (deg.)]:"; ExternalControl "External control of PQ"; NpNq "Parameters [ np  nq ]:"; TimeConstants "Time constants [Tp1 Tp2 Tq1 Tq2]  (s):"; MinimumVoltage "Minimum voltage Vmin (pu):"; LoadFlowParameters "Load Flow parameters"
      mask help:
      | Implements a single-phase dynamic load. Active  power P and reactive
      | power Q absorbed by the load vary as function of voltage V  according to the
      | following equations:
      |
      |   If V>Vmin, P and Q vary as follows:
      |        P = Po * (V/Vo)^np * (1+Tp1.s)/(1+Tp2.s)
      |        Q = Qo * (V/Vo)^nq * (1+Tq1.s)/(1+Tq2.s)
      |   if V<Vmin
      |      Same equations with np=nq=2 (constant impedance load)
      mask init: same as ng_pv_dynamic_dbus_p_1_sm_ng/SM_NG/Single-Phase Dynamic Load32
      mask Help: helpview(psbhelp)
      mask Callback ExternalControl: powericon('ThreePhaseDynamicLoadCback',gcb);
      mask Display:
      | plot(.2*[0 3.5 5 2 0], .2*[1 1 4.5 4.5 1])
      | plot(.2*[1.7 3.5], .2*[1 4.5])
      | plot(.2*[1.1 4.3], .2*[3 3])
      | plot(.2*[.6 3.9], .2*[2 2])
      | plot(.2*[1.7 4.7], .2*[3.9 3.9])
  Single-Phase Dynamic Load55 : Subsystem  DialogController=POWERSYS.PowerSysDialog  mask(Single-Phase Dynamic Load){NominalVoltage=[7967.43 60 ], ActiveReactivePowers=[-92428.700 13104.122], PositiveSequence=[1 0], ExternalControl=on, NpNq=[np nq], TimeConstants=[0  0  0  0], MinimumVoltage=Vmin, LoadFlowParameters=[4,0,0,0,0]}
      mask prompts: NominalVoltage "Nominal voltage and frequency  [Vn(Vrms) fn(Hz)]:"; ActiveReactivePowers "Active and reactive power at initial voltage [Po(W) Qo(var)]:"; PositiveSequence "Initial voltage Vo [Mag(pu) Phase (deg.)]:"; ExternalControl "External control of PQ"; NpNq "Parameters [ np  nq ]:"; TimeConstants "Time constants [Tp1 Tp2 Tq1 Tq2]  (s):"; MinimumVoltage "Minimum voltage Vmin (pu):"; LoadFlowParameters "Load Flow parameters"
      mask help:
      | Implements a single-phase dynamic load. Active  power P and reactive
      | power Q absorbed by the load vary as function of voltage V  according to the
      | following equations:
      |
      |   If V>Vmin, P and Q vary as follows:
      |        P = Po * (V/Vo)^np * (1+Tp1.s)/(1+Tp2.s)
      |        Q = Qo * (V/Vo)^nq * (1+Tq1.s)/(1+Tq2.s)
      |   if V<Vmin
      |      Same equations with np=nq=2 (constant impedance load)
      mask init: same as ng_pv_dynamic_dbus_p_1_sm_ng/SM_NG/Single-Phase Dynamic Load32
      mask Help: helpview(psbhelp)
      mask Callback ExternalControl: powericon('ThreePhaseDynamicLoadCback',gcb);
      mask Display:
      | plot(.2*[0 3.5 5 2 0], .2*[1 1 4.5 4.5 1])
      | plot(.2*[1.7 3.5], .2*[1 4.5])
      | plot(.2*[1.1 4.3], .2*[3 3])
      | plot(.2*[.6 3.9], .2*[2 2])
      | plot(.2*[1.7 4.7], .2*[3.9 3.9])
  Single-Phase Dynamic Load56 : Subsystem  DialogController=POWERSYS.PowerSysDialog  mask(Single-Phase Dynamic Load){NominalVoltage=|, ActiveReactivePowers=[-58997.800 8411.427], PositiveSequence=[1 0], ExternalControl=on, NpNq=[np nq], TimeConstants=[0  0  0  0], MinimumVoltage=Vmin, LoadFlowParameters=[4,0,0,0,0]}
      mask NominalVoltage=|
      | [7967.43
      | 60]
      mask prompts: NominalVoltage "Nominal voltage and frequency  [Vn(Vrms) fn(Hz)]:"; ActiveReactivePowers "Active and reactive power at initial voltage [Po(W) Qo(var)]:"; PositiveSequence "Initial voltage Vo [Mag(pu) Phase (deg.)]:"; ExternalControl "External control of PQ"; NpNq "Parameters [ np  nq ]:"; TimeConstants "Time constants [Tp1 Tp2 Tq1 Tq2]  (s):"; MinimumVoltage "Minimum voltage Vmin (pu):"; LoadFlowParameters "Load Flow parameters"
      mask help:
      | Implements a single-phase dynamic load. Active  power P and reactive
      | power Q absorbed by the load vary as function of voltage V  according to the
      | following equations:
      |
      |   If V>Vmin, P and Q vary as follows:
      |        P = Po * (V/Vo)^np * (1+Tp1.s)/(1+Tp2.s)
      |        Q = Qo * (V/Vo)^nq * (1+Tq1.s)/(1+Tq2.s)
      |   if V<Vmin
      |      Same equations with np=nq=2 (constant impedance load)
      mask init: same as ng_pv_dynamic_dbus_p_1_sm_ng/SM_NG/Single-Phase Dynamic Load32
      mask Help: helpview(psbhelp)
      mask Callback ExternalControl: powericon('ThreePhaseDynamicLoadCback',gcb);
      mask Display:
      | plot(.2*[0 3.5 5 2 0], .2*[1 1 4.5 4.5 1])
      | plot(.2*[1.7 3.5], .2*[1 4.5])
      | plot(.2*[1.1 4.3], .2*[3 3])
      | plot(.2*[.6 3.9], .2*[2 2])
      | plot(.2*[1.7 4.7], .2*[3.9 3.9])
  Single-Phase Dynamic Load57 : Subsystem  DialogController=POWERSYS.PowerSysDialog  mask(Single-Phase Dynamic Load){NominalVoltage=[7967.43 60 ], ActiveReactivePowers=[-368952.000 56486.553], PositiveSequence=[1 0], ExternalControl=on, NpNq=[np nq], TimeConstants=[0  0  0  0], MinimumVoltage=Vmin, LoadFlowParameters=[4,0,0,0,0]}
      mask prompts: NominalVoltage "Nominal voltage and frequency  [Vn(Vrms) fn(Hz)]:"; ActiveReactivePowers "Active and reactive power at initial voltage [Po(W) Qo(var)]:"; PositiveSequence "Initial voltage Vo [Mag(pu) Phase (deg.)]:"; ExternalControl "External control of PQ"; NpNq "Parameters [ np  nq ]:"; TimeConstants "Time constants [Tp1 Tp2 Tq1 Tq2]  (s):"; MinimumVoltage "Minimum voltage Vmin (pu):"; LoadFlowParameters "Load Flow parameters"
      mask help:
      | Implements a single-phase dynamic load. Active  power P and reactive
      | power Q absorbed by the load vary as function of voltage V  according to the
      | following equations:
      |
      |   If V>Vmin, P and Q vary as follows:
      |        P = Po * (V/Vo)^np * (1+Tp1.s)/(1+Tp2.s)
      |        Q = Qo * (V/Vo)^nq * (1+Tq1.s)/(1+Tq2.s)
      |   if V<Vmin
      |      Same equations with np=nq=2 (constant impedance load)
      mask init: same as ng_pv_dynamic_dbus_p_1_sm_ng/SM_NG/Single-Phase Dynamic Load32
      mask Help: helpview(psbhelp)
      mask Callback ExternalControl: powericon('ThreePhaseDynamicLoadCback',gcb);
      mask Display:
      | plot(.2*[0 3.5 5 2 0], .2*[1 1 4.5 4.5 1])
      | plot(.2*[1.7 3.5], .2*[1 4.5])
      | plot(.2*[1.1 4.3], .2*[3 3])
      | plot(.2*[.6 3.9], .2*[2 2])
      | plot(.2*[1.7 4.7], .2*[3.9 3.9])
  Single-Phase Dynamic Load58 : Subsystem  DialogController=POWERSYS.PowerSysDialog  mask(Single-Phase Dynamic Load){NominalVoltage=|, ActiveReactivePowers=|, PositiveSequence=[1 0], ExternalControl=on, NpNq=[np nq], TimeConstants=[0  0  0  0], MinimumVoltage=Vmin, LoadFlowParameters=[4,0,0,0,0]}
      mask NominalVoltage=|
      | [7967.43
      | 60 ]
      mask ActiveReactivePowers=|
      | [-331064.000
      |  50291.023]
      mask prompts: NominalVoltage "Nominal voltage and frequency  [Vn(Vrms) fn(Hz)]:"; ActiveReactivePowers "Active and reactive power at initial voltage [Po(W) Qo(var)]:"; PositiveSequence "Initial voltage Vo [Mag(pu) Phase (deg.)]:"; ExternalControl "External control of PQ"; NpNq "Parameters [ np  nq ]:"; TimeConstants "Time constants [Tp1 Tp2 Tq1 Tq2]  (s):"; MinimumVoltage "Minimum voltage Vmin (pu):"; LoadFlowParameters "Load Flow parameters"
      mask help:
      | Implements a single-phase dynamic load. Active  power P and reactive
      | power Q absorbed by the load vary as function of voltage V  according to the
      | following equations:
      |
      |   If V>Vmin, P and Q vary as follows:
      |        P = Po * (V/Vo)^np * (1+Tp1.s)/(1+Tp2.s)
      |        Q = Qo * (V/Vo)^nq * (1+Tq1.s)/(1+Tq2.s)
      |   if V<Vmin
      |      Same equations with np=nq=2 (constant impedance load)
      mask init: same as ng_pv_dynamic_dbus_p_1_sm_ng/SM_NG/Single-Phase Dynamic Load32
      mask Help: helpview(psbhelp)
      mask Callback ExternalControl: powericon('ThreePhaseDynamicLoadCback',gcb);
      mask Display:
      | plot(.2*[0 3.5 5 2 0], .2*[1 1 4.5 4.5 1])
      | plot(.2*[1.7 3.5], .2*[1 4.5])
      | plot(.2*[1.1 4.3], .2*[3 3])
      | plot(.2*[.6 3.9], .2*[2 2])
      | plot(.2*[1.7 4.7], .2*[3.9 3.9])
  Single-Phase Dynamic Load59 : Subsystem  DialogController=POWERSYS.PowerSysDialog  mask(Single-Phase Dynamic Load){NominalVoltage=|, ActiveReactivePowers=|, PositiveSequence=[1 0], ExternalControl=on, NpNq=[np nq], TimeConstants=[0  0  0  0], MinimumVoltage=Vmin, LoadFlowParameters=[4,0,0,0,0]}
      mask NominalVoltage=|
      | [7967.43
      | 60 ]
      mask ActiveReactivePowers=|
      | [-340231.000
      | 51005.605]
      mask prompts: NominalVoltage "Nominal voltage and frequency  [Vn(Vrms) fn(Hz)]:"; ActiveReactivePowers "Active and reactive power at initial voltage [Po(W) Qo(var)]:"; PositiveSequence "Initial voltage Vo [Mag(pu) Phase (deg.)]:"; ExternalControl "External control of PQ"; NpNq "Parameters [ np  nq ]:"; TimeConstants "Time constants [Tp1 Tp2 Tq1 Tq2]  (s):"; MinimumVoltage "Minimum voltage Vmin (pu):"; LoadFlowParameters "Load Flow parameters"
      mask help:
      | Implements a single-phase dynamic load. Active  power P and reactive
      | power Q absorbed by the load vary as function of voltage V  according to the
      | following equations:
      |
      |   If V>Vmin, P and Q vary as follows:
      |        P = Po * (V/Vo)^np * (1+Tp1.s)/(1+Tp2.s)
      |        Q = Qo * (V/Vo)^nq * (1+Tq1.s)/(1+Tq2.s)
      |   if V<Vmin
      |      Same equations with np=nq=2 (constant impedance load)
      mask init: same as ng_pv_dynamic_dbus_p_1_sm_ng/SM_NG/Single-Phase Dynamic Load32
      mask Help: helpview(psbhelp)
      mask Callback ExternalControl: powericon('ThreePhaseDynamicLoadCback',gcb);
      mask Display:
      | plot(.2*[0 3.5 5 2 0], .2*[1 1 4.5 4.5 1])
      | plot(.2*[1.7 3.5], .2*[1 4.5])
      | plot(.2*[1.1 4.3], .2*[3 3])
      | plot(.2*[.6 3.9], .2*[2 2])
      | plot(.2*[1.7 4.7], .2*[3.9 3.9])
  Single-Phase Dynamic Load60 : Subsystem  DialogController=POWERSYS.PowerSysDialog  mask(Single-Phase Dynamic Load){NominalVoltage=|, ActiveReactivePowers=[-57081.600 8327.905], PositiveSequence=[1 0], ExternalControl=on, NpNq=[np nq], TimeConstants=[0  0  0  0], MinimumVoltage=Vmin, LoadFlowParameters=[4,0,0,0,0]}
      mask NominalVoltage=|
      | [7967.43
      | 60]
      mask prompts: NominalVoltage "Nominal voltage and frequency  [Vn(Vrms) fn(Hz)]:"; ActiveReactivePowers "Active and reactive power at initial voltage [Po(W) Qo(var)]:"; PositiveSequence "Initial voltage Vo [Mag(pu) Phase (deg.)]:"; ExternalControl "External control of PQ"; NpNq "Parameters [ np  nq ]:"; TimeConstants "Time constants [Tp1 Tp2 Tq1 Tq2]  (s):"; MinimumVoltage "Minimum voltage Vmin (pu):"; LoadFlowParameters "Load Flow parameters"
      mask help:
      | Implements a single-phase dynamic load. Active  power P and reactive
      | power Q absorbed by the load vary as function of voltage V  according to the
      | following equations:
      |
      |   If V>Vmin, P and Q vary as follows:
      |        P = Po * (V/Vo)^np * (1+Tp1.s)/(1+Tp2.s)
      |        Q = Qo * (V/Vo)^nq * (1+Tq1.s)/(1+Tq2.s)
      |   if V<Vmin
      |      Same equations with np=nq=2 (constant impedance load)
      mask init: same as ng_pv_dynamic_dbus_p_1_sm_ng/SM_NG/Single-Phase Dynamic Load32
      mask Help: helpview(psbhelp)
      mask Callback ExternalControl: powericon('ThreePhaseDynamicLoadCback',gcb);
      mask Display:
      | plot(.2*[0 3.5 5 2 0], .2*[1 1 4.5 4.5 1])
      | plot(.2*[1.7 3.5], .2*[1 4.5])
      | plot(.2*[1.1 4.3], .2*[3 3])
      | plot(.2*[.6 3.9], .2*[2 2])
      | plot(.2*[1.7 4.7], .2*[3.9 3.9])
  Subsystem : Subsystem
  TSync PCIe Ctrl1 : rtio_spectracom/TSync PCIe Ctrl  devIx=0  holdover_timeout=5  timestamp_en=on  set_time_en=off  ts_wo_sync_opt=Simulation time
  Terminator1 : Terminator
  Terminator3 : Terminator
  Three-Phase Transformer (Two Windings)2 : powerlib/Elements/Three-Phase Transformer (Two Windings)  Winding1Connection=Yg  Winding2Connection=Yg  CoreType=Three single-phase transformers  SetSaturation=off  Hysteresis=off  DataFile='hysteresis'  SetInitialFlux=off  Measurements=None  UNITS=pu  NominalPower=[9990e3 , 60 ]  Winding1=[13.8e3 , 0.0001, 0.001]  Winding2=[13.8e3, 0.0001, 0.001]  Rm=4000  Lm=inf  L0=0.5  Saturation=[ 0,0 ; 0.0024,1.2 ; 1.0,1.52 ]  InitialFluxes=[ 0.8 , -0.8 , 0.7 ]  MoreParameters=off  BreakLoop=off  DataType=off  TransfoNumber=1
  Three-Phase Source1 : powerlib/Electrical Sources/Three-Phase Source  InternalConnection=Yg  VoltagePhases=off  Voltage=13800*1.02  PhaseAngle=0  Voltage_phases=[25e3 25e3 25e3]/sqrt(3)  PhaseAngles_phases=[0 -120 +120]  Frequency=60  NonIdealSource=on  SpecifyImpedance=off  Resistance=0.0339  Inductance=(1.0783)/(377)  ShortCircuitLevel=2e6  BaseVoltage=13.8e3  XRratio=4  BusType=swing  Pref=0  Qref=0  Prefabc=[10e3, 10e3, 10e3]  Qrefabc=[0, 0, 0]  Qmin=-inf  Qmax=inf
  Timestamp selector : Subsystem
  rtlab_send_subsystem : Subsystem  Priority=-100
      mask Display: text(0,0,'');
  zzzOpComm : Subsystem
      mask init:
      | opmaskdisplay('maskdisplay_block',gcb,'disp(''OpComm'')');
      mask Display:
      | patch([0 0.5 0.7 0],[1 1 0 0],[0.7 0.75 0.9]);
      | patch([1 0.53 0.73 1],[1 1 0 0],[1 0.8 0.7]);
      | plot([0 0 1 1 0],[0 1 1 0 0]);
      | disp('OpComm')
  tag scope: rtlab_send_1=global, rtlab_send_2=global, rtlab_send_3=global, rtlab_send_4=global, rtlab_send_5=global, rtlab_send_6=global
  wires:
  Clock1/1 -> Real Power/1, Real Power1/1
  Real Power/1 -> [P]
  Real Power1/1 -> [Q]
  [PPV842A] -> Mux4/1
  [QPV842A] -> Mux4/2
  Mux4/1 -> [PQPV842A]
  [PPV842B] -> Mux3/1
  [QPV842B] -> Mux3/2
  Mux3/1 -> [PQPV842B]
  [PPV842C] -> Mux2/1
  [QPV842C] -> Mux2/2
  Mux2/1 -> [PQPV842C]
  [PPV838A] -> Mux1/1
  [QPV838A] -> Mux1/2
  Mux1/1 -> [PQPV838A]
  OpMonitor/1 -> [rtlab_send_1]
  [PPV1] -> Mux/1
  [QPV1] -> Mux/2
  Mux/1 -> [PQPV1]
  [PPV872A] -> Mux8/1
  [QPV872A] -> Mux8/2
  Mux8/1 -> [PQPV872A]
  [PPV872B] -> Mux7/1
  [QPV872B] -> Mux7/2
  Mux7/1 -> [PQPV872B]
  [PPV872C] -> Mux6/1
  [QPV872C] -> Mux6/2
  Mux6/1 -> [PQPV872C]
  [PPV857A] -> Mux11/1
  [QPV857A] -> Mux11/2
  Mux11/1 -> [PQPV857A]
  [PPV857B] -> Mux10/1
  [QPV857B] -> Mux10/2
  Mux10/1 -> [PQPV857B]
  [PPV857C] -> Mux9/1
  [QPV857C] -> Mux9/2
  Mux9/1 -> [PQPV857C]
  [PPV854A] -> Mux14/1
  [QPV854A] -> Mux14/2
  Mux14/1 -> [PQPV854A]
  [PPV854B] -> Mux13/1
  [QPV854B] -> Mux13/2
  Mux13/1 -> [PQPV854B]
  [PPV854C] -> Mux12/1
  [QPV854C] -> Mux12/2
  Mux12/1 -> [PQPV854C]
  Mux22/1 -> [PQPV866A]
  Mux21/1 -> [PQPV866B]
  Mux20/1 -> [PQPV866C]
  [PPV845A] -> Mux25/1
  [QPV845A] -> Mux25/2
  Mux25/1 -> [PQPV845A]
  [PPV845B] -> Mux24/1
  [QPV845B] -> Mux24/2
  Mux24/1 -> [PQPV845B]
  [PPV845C] -> Mux23/1
  [QPV845C] -> Mux23/2
  Mux23/1 -> [PQPV845C]
  [PPV860A] -> Mux16/1
  [QPV860A] -> Mux16/2
  Mux16/1 -> [PQPV860A]
  [PPV860B] -> Mux15/1
  [QPV860B] -> Mux15/2
  Mux15/1 -> [PQPV860B]
  [PPV860C] -> Mux26/1
  [QPV860C] -> Mux26/2
  Mux26/1 -> [PQPV860C]
  [PPV863A] -> Mux19/1
  [QPV863A] -> Mux19/2
  Mux19/1 -> [PQPV863A]
  [PPV863B] -> Mux18/1
  [QPV863B] -> Mux18/2
  Mux18/1 -> [PQPV863B]
  [PPV863C] -> Mux17/1
  [QPV863C] -> Mux17/2
  Mux17/1 -> [PQPV863C]
  [PPV866A] -> Mux22/1
  [QPV866A] -> Mux22/2
  [PPV866B] -> Mux21/1
  [QPV866B] -> Mux21/2
  [PPV866C] -> Mux20/1
  [QPV866C] -> Mux20/2
  [PPV848A] -> Mux29/1
  Mux29/1 -> [PQPV848A]
  Mux28/1 -> [PQPV848B]
  Mux27/1 -> [PQPV848C]
  [QPV848C] -> Mux27/2
  [PPV848C] -> Mux27/1
  [QPV848B] -> Mux28/2
  [PPV848B] -> Mux28/1
  [QPV848A] -> Mux29/2
  [PPV851A] -> Mux30/1
  Mux30/1 -> [PQPV851A]
  [QPV851A] -> Mux30/2
  [PPV869A] -> Mux31/1
  Mux31/1 -> [PQPV869A]
  [QPV869A] -> Mux31/2
  [V_IED11] -> PLL (3ph)2/1, RMS2/1, Mux5/1
  [V_IED3] -> Selector11/1, Selector10/1, Selector9/1
  [V_IED4] -> Selector14/1, Selector13/1, Selector12/1
  [V_IED5A] -> Selector17/1, Selector16/1, Selector15/1
  [V_IED6A] -> Selector20/1, Selector19/1, Selector18/1
  [V_IED8] -> Selector23/1, Selector22/1, Selector21/1
  [V_IED9] -> Selector26/1, Selector25/1, Selector24/1
  [V_IED13A] -> Selector32/1, Selector31/1, Selector30/1
  [V_IED2A] -> Selector6/1, Selector8/1, Selector7/1
  [V_IED12A] -> Selector29/1, Selector28/1, Selector27/1
  Demux1/1 -> [PPV1]
  Demux1/2 -> [QPV1]
  Demux1/3 -> [PPV851A]
  Demux1/4 -> [QPV851A]
  RMS28/1 -> [rtlab_send_2]
  PLL (3ph)2/1 -> [freq]
  [freq] -> Mux5/2
  [V_IED7A] -> Mux5/3
  [freq] -> Mux5/4
  [V_IED10] -> Mux5/5
  [freq] -> Mux5/6
  [V_IED14A] -> Mux5/7
  [freq] -> Mux5/8
  Selector6/1 -> Mux5/9
  [freq] -> Mux5/10
  Selector7/1 -> Mux5/11
  [freq] -> Mux5/12
  Selector8/1 -> Mux5/13
  [freq] -> Mux5/14
  Demux1/5 -> [PPV838A]
  Demux1/6 -> [QPV838A]
  Demux1/7 -> [PPV869A]
  Demux1/8 -> [QPV869A]
  Demux1/9 -> [PPV857A]
  Demux1/10 -> [QPV857A]
  Demux1/11 -> [PPV857B]
  Demux1/12 -> [QPV857B]
  Demux1/13 -> [PPV857C]
  Demux1/14 -> [QPV857C]
  Demux1/15 -> [PPV872A]
  Demux1/16 -> [QPV872A]
  Demux1/17 -> [PPV872B]
  Demux1/18 -> [QPV872B]
  Demux1/19 -> [PPV872C]
  Demux1/20 -> [QPV872C]
  RMS2/1 -> Display/1
  Demux1/62 -> [QPV866C]
  Demux1/61 -> [PPV866C]
  Demux1/60 -> [QPV866B]
  Demux1/59 -> [PPV866B]
  Demux1/58 -> [QPV866A]
  Demux1/57 -> [PPV866A]
  Demux1/56 -> [QPV860C]
  Demux1/55 -> [PPV860C]
  Demux1/54 -> [QPV860B]
  Demux1/53 -> [PPV860B]
  Demux1/52 -> [QPV860A]
  Demux1/51 -> [PPV860A]
  Demux1/50 -> [QPV842C]
  Demux1/49 -> [PPV842C]
  Demux1/48 -> [QPV842B]
  Demux1/47 -> [PPV842B]
  Demux1/46 -> [QPV842A]
  Demux1/45 -> [PPV842A]
  Demux1/44 -> [QPV854C]
  Demux1/43 -> [PPV854C]
  Demux1/42 -> [QPV854B]
  Demux1/41 -> [PPV854B]
  Demux1/40 -> [QPV854A]
  Demux1/39 -> [PPV854A]
  Demux1/38 -> [QPV845C]
  Demux1/37 -> [PPV845C]
  Demux1/36 -> [QPV845B]
  Demux1/35 -> [PPV845B]
  Demux1/21 -> [PPV848A]
  Demux1/22 -> [QPV848A]
  Demux1/23 -> [PPV848B]
  Demux1/24 -> [QPV848B]
  Demux1/25 -> [PPV848C]
  Demux1/26 -> [QPV848C]
  Demux1/27 -> [PPV863A]
  Demux1/28 -> [QPV863A]
  Demux1/29 -> [PPV863B]
  Demux1/30 -> [QPV863B]
  Demux1/31 -> [PPV863C]
  Demux1/32 -> [QPV863C]
  Demux1/33 -> [PPV845A]
  Demux1/34 -> [QPV845A]
  zzzOpComm/1(Out1) -> Demux1/1
  Mux5/1 -> RMS28/1
  Selector9/1 -> Mux5/15
  [freq] -> Mux5/16
  Selector10/1 -> Mux5/17
  [freq] -> Mux5/18
  Selector11/1 -> Mux5/19
  [freq] -> Mux5/20
  Selector12/1 -> Mux5/21
  [freq] -> Mux5/22
  Selector13/1 -> Mux5/23
  [freq] -> Mux5/24
  Selector14/1 -> Mux5/25
  [freq] -> Mux5/26
  Selector15/1 -> Mux5/27
  [freq] -> Mux5/28
  Selector16/1 -> Mux5/29
  [freq] -> Mux5/30
  Selector17/1 -> Mux5/31
  [freq] -> Mux5/32
  Selector18/1 -> Mux5/33
  [freq] -> Mux5/34
  Selector19/1 -> Mux5/35
  [freq] -> Mux5/36
  Selector20/1 -> Mux5/37
  [freq] -> Mux5/38
  Selector21/1 -> Mux5/39
  [freq] -> Mux5/40
  Selector22/1 -> Mux5/41
  [freq] -> Mux5/42
  Selector23/1 -> Mux5/43
  [freq] -> Mux5/44
  Selector24/1 -> Mux5/45
  [freq] -> Mux5/46
  Selector25/1 -> Mux5/47
  [freq] -> Mux5/48
  Selector26/1 -> Mux5/49
  [freq] -> Mux5/50
  Selector27/1 -> Mux5/51
  [freq] -> Mux5/52
  Selector28/1 -> Mux5/53
  [freq] -> Mux5/54
  Selector29/1 -> Mux5/55
  [freq] -> Mux5/56
  Selector30/1 -> Mux5/57
  [freq] -> Mux5/58
  Selector31/1 -> Mux5/59
  [freq] -> Mux5/60
  Selector32/1 -> Mux5/61
  [freq] -> Mux5/62
  [PQPV863A] -> Single-Phase Dynamic Load60/1(PQ)
  [PQPV863B] -> Single-Phase Dynamic Load32/1(PQ)
  [PQPV863C] -> Single-Phase Dynamic Load33/1(PQ)
  [PQPV866A] -> Single-Phase Dynamic Load34/1(PQ)
  [PQPV866B] -> Single-Phase Dynamic Load35/1(PQ)
  [PQPV866C] -> Single-Phase Dynamic Load36/1(PQ)
  [PQPV857A] -> Single-Phase Dynamic Load44/1(PQ)
  [PQPV857B] -> Single-Phase Dynamic Load45/1(PQ)
  [PQPV857C] -> Single-Phase Dynamic Load46/1(PQ)
  [PQPV860A] -> Single-Phase Dynamic Load57/1(PQ)
  [PQPV860B] -> Single-Phase Dynamic Load58/1(PQ)
  [PQPV860C] -> Single-Phase Dynamic Load59/1(PQ)
  [PQPV845A] -> Single-Phase Dynamic Load37/1(PQ)
  [PQPV845B] -> Single-Phase Dynamic Load38/1(PQ)
  [PQPV845C] -> Single-Phase Dynamic Load39/1(PQ)
  [PQPV869A] -> Single-Phase Dynamic Load53/1(PQ)
  [PQPV851A] -> Single-Phase Dynamic Load55/1(PQ)
  [PQPV872A] -> Single-Phase Dynamic Load40/1(PQ)
  [PQPV872B] -> Single-Phase Dynamic Load41/1(PQ)
  [PQPV872C] -> Single-Phase Dynamic Load43/1(PQ)
  [PQPV838A] -> Single-Phase Dynamic Load54/1(PQ)
  [PQPV842A] -> Single-Phase Dynamic Load50/1(PQ)
  [PQPV842B] -> Single-Phase Dynamic Load51/1(PQ)
  [PQPV842C] -> Single-Phase Dynamic Load52/1(PQ)
  [P] -> Dynamic Load BCDC2/1(P)
  [Q] -> Dynamic Load BCDC2/2(Q)
  [P] -> Dynamic Load BCDC1/1(P)
  [Q] -> Dynamic Load BCDC1/2(Q)
  [P] -> Dynamic Load BCDC3/1(P)
  [Q] -> Dynamic Load BCDC3/2(Q)
  [PQPV848A] -> Single-Phase Dynamic Load30/1(PQ)
  [PQPV848B] -> Single-Phase Dynamic Load42/1(PQ)
  [PQPV848C] -> Single-Phase Dynamic Load56/1(PQ)
  [PQPV854C] -> Single-Phase Dynamic Load49/1(PQ)
  [PQPV854B] -> Single-Phase Dynamic Load48/1(PQ)
  [PQPV854A] -> Single-Phase Dynamic Load47/1(PQ)
  [PQPV1] -> PV11/1(PQ)
  [V_IED1] -> Mux44/1
  [I_IED1] -> Mux44/2
  [V_IED2] -> Mux45/1
  [I_IED2] -> Mux45/2
  [V_IED3] -> Mux46/1
  [I_IED3] -> Mux46/2
  [V_IED5] -> Mux48/1
  [I_IED5] -> Mux48/2
  [V_IED6] -> Mux32/1
  [I_IED6] -> Mux32/2
  [V_IED7] -> Mux33/1
  [I_IED7] -> Mux33/2
  [V_IED8] -> Mux34/1
  [I_IED8] -> Mux34/2
  [V_IED10] -> Mux35/1
  [I_IED10] -> Mux35/2
  [V_IED11] -> Mux36/1
  [I_IED11] -> Mux36/2
  [V_IED12A] -> Mux37/1
  [I_IED12A] -> Mux37/2
  [V_IED13] -> Mux38/1
  [I_IED13] -> Mux38/2
  [V_IED14] -> Mux39/1
  [I_IED14] -> Mux39/2
  [V_IED15] -> Mux40/1
  [I_IED15] -> Mux40/2
  [V_IED9] -> Mux41/1
  [I_IED9] -> Mux41/2
  Bus Creator/1 -> [rtlab_send_3]
  [V_IED4] -> Mux47/1
  [I_IED4] -> Mux47/2
  Constant8/1 -> TSync PCIe Ctrl1/1
  Timestamp selector/1(ts_out) -> [rtlab_send_4]
  TSync PCIe Ctrl1/1 -> [rtlab_send_5], Timestamp selector/1(ts_in)
  [I_IED7A] -> Mux42/2
  [V_IED7A] -> Mux42/1
  [I_IED6A] -> Mux43/2
  [V_IED6A] -> Mux43/1
  [I_IED2A] -> Mux49/2
  [V_IED2A] -> Mux49/1
  [V_IED12] -> Mux50/1
  [I_IED12] -> Mux50/2
  [V_IED13A] -> Mux51/1
  [I_IED13A] -> Mux51/2
  [V_IED14A] -> Mux52/1
  [I_IED14A] -> Mux52/2
  Mux40/1 -> Bus Creator/22
  Mux36/1 -> Bus Creator/15
  Mux50/1 -> Bus Creator/16
  Mux37/1 -> Bus Creator/17
  Mux38/1 -> Bus Creator/18
  Mux51/1 -> Bus Creator/19
  Mux39/1 -> Bus Creator/20
  Mux52/1 -> Bus Creator/21
  Mux35/1 -> Bus Creator/14
  Mux41/1 -> Bus Creator/13
  Mux34/1 -> Bus Creator/12
  Mux42/1 -> Bus Creator/11
  Mux33/1 -> Bus Creator/10
  Mux43/1 -> Bus Creator/9
  Mux32/1 -> Bus Creator/8
  Mux48/1 -> Bus Creator/6
  Mux47/1 -> Bus Creator/5
  Mux46/1 -> Bus Creator/4
  Mux44/1 -> Bus Creator/1
  Mux45/1 -> Bus Creator/2
  Mux49/1 -> Bus Creator/3
  [V_IED5A] -> Mux53/1
  [I_IED5A] -> Mux53/2
  Mux53/1 -> Bus Creator/7
  [V_IED15] -> RMS/1
  RMS/1 -> Display1/1
  OpCtrl ML605EX1/1 -> Terminator1/1
  OpCtrl ML605EX1/2 -> Terminator3/1
  Mux54/1 -> [rtlab_send_6]
  Subsystem/1(Out1) -> Mux54/1
  Subsystem/2(Out2) -> Mux54/2
  Subsystem/3(Out3) -> Mux54/3
  [V_IED15] -> RMS3/1
  RMS3/1 -> Divide/1
  Divide/1 -> Dynamic load measurement output1/1
  Constant/1 -> Divide/2
  connections:
  IED6A/LConn1 -- IED6/LConn1 -- Series  Load63/LConn1 -- Line777/LConn1 -- Line775A/LConn1 -- Line425/RConn1
  Line425/RConn2 -- Line775A/LConn2 -- IED6A/LConn2 -- IED6/LConn2 -- Series  Load64/LConn1 -- Line777/LConn2
  Line775A/LConn3 -- Line425/RConn3 -- Series  Load61/LConn1 -- Line777/LConn3 -- IED6/LConn3 -- IED6A/LConn3
  Line405B/RConn2 -- IED5A/LConn2 -- IED5/LConn2 -- Line809/LConn2 -- Dynamic Load BCDC2/RConn2
  Line405B/RConn1 -- IED5A/LConn1 -- IED5/LConn1 -- Line809/LConn1 -- Dynamic Load BCDC2/RConn1
  Line405B/RConn3 -- IED5A/LConn3 -- IED5/LConn3 -- Line809/LConn3 -- Dynamic Load BCDC2/RConn3
  IED11/LConn2 -- Line687/RConn2 -- Series  Load75/LConn1 -- Line718A/LConn2
  IED11/LConn1 -- Line687/RConn1 -- Series  Load74/LConn1 -- Line718A/LConn1
  IED11/LConn3 -- Line687/RConn3 -- Series  Load72/LConn1 -- Line718A/LConn3
  Line718B/RConn3 -- IED2A/LConn3 -- Dynamic Load BCDC1/RConn3 -- Line369/LConn3 -- IED2/LConn3
  Line718B/RConn2 -- IED2A/LConn2 -- Dynamic Load BCDC1/RConn2 -- Line369/LConn2 -- IED2/LConn2
  IED2A/LConn1 -- Line718B/RConn1 -- Dynamic Load BCDC1/RConn1 -- Line369/LConn1 -- IED2/LConn1
  IED9/LConn2 -- Series  Load100/LConn1 -- Line491/RConn2
  IED9/LConn3 -- Line491/RConn3 -- Series  Load98/LConn1 -- Line614/LConn1
  IED9/LConn1 -- Series  Load99/LConn1 -- Line491/RConn1
  IED4/LConn2 -- Series  Load97/LConn1 -- Line405A/LConn2 -- Line425/LConn2 -- Line489/RConn2
  IED8/LConn3 -- Line687/LConn3 -- Dynamic Load BCDC3/RConn3 -- Line491/LConn3 -- Line775B/RConn3
  IED8/LConn2 -- Line687/LConn2 -- Dynamic Load BCDC3/RConn2 -- Line491/LConn2 -- Line775B/RConn2
  IED8/LConn1 -- Line687/LConn1 -- Dynamic Load BCDC3/RConn1 -- Line491/LConn1 -- Line775B/RConn1
  IED4/LConn1 -- Series  Load86/LConn1 -- Line405A/LConn1 -- Line425/LConn1 -- Line489/RConn1
  Line937/RConn1 -- IED7A/RConn1 -- Series  Load62/LConn1 -- Line489/LConn1 -- IED7/LConn1
  Line937/RConn2 -- Series  Load71/LConn1 -- Line489/LConn2 -- IED7/LConn2
  Line937/RConn3 -- Series  Load28/LConn1 -- Line489/LConn3 -- IED7/LConn3
  IED13A/LConn1 -- Series  Load95/LConn1 -- Series  Load8/LConn1 -- IED13/LConn1
  IED13A/LConn2 -- Series  Load96/LConn1 -- Series  Load9/LConn1 -- IED13/LConn2
  Series  Load94/LConn1 -- IED13A/LConn3 -- Series  Load7/LConn1 -- IED13/LConn3
  IED12A/LConn1 -- IED12/LConn1 -- Series  Load23/LConn1 -- Line777/RConn1
  IED12A/LConn2 -- IED12/LConn2 -- Series  Load24/LConn1 -- Line777/RConn2
  IED12A/LConn3 -- IED12/LConn3 -- Series  Load22/LConn1 -- Line777/RConn3
  IED3/LConn1 -- Series  Load77/LConn1 -- Line369/RConn1
  IED3/LConn2 -- Series  Load79/LConn1 -- Line369/RConn2
  IED3/LConn3 -- Series  Load76/LConn1 -- Line369/RConn3
  Series  Load60/RConn1 -- Ground42/LConn1 -- Series  Load42/RConn1 -- Series  Load80/RConn1
  Series  Load82/RConn1 -- Ground43/LConn1 -- Series  Load81/RConn1 -- Series  Load83/RConn1
  Series  Load85/RConn1 -- Ground45/LConn1 -- Series  Load84/RConn1 -- Series  Load87/RConn1
  Series  Load89/RConn1 -- Ground46/LConn1 -- Series  Load88/RConn1 -- Series  Load90/RConn1
  Series  Load93/RConn1 -- Ground47/LConn1 -- Series  Load91/RConn1 -- Series  Load92/RConn1
  Series  Load96/RConn1 -- Ground48/LConn1 -- Series  Load94/RConn1 -- Series  Load95/RConn1
  Line489/RConn3 -- Line425/LConn3 -- Series  Load78/LConn1 -- Line405A/LConn3 -- IED4/LConn3
  Series  Load71/RConn1 -- Series  Load62/RConn1 -- Ground10/LConn1 -- Series  Load28/RConn1
  Series  Load97/RConn1 -- Series  Load86/RConn1 -- Ground44/LConn1 -- Series  Load78/RConn1
  Series  Load75/RConn1 -- Ground16/LConn1 -- Series  Load74/RConn1 -- Series  Load72/RConn1
  Series  Load63/RConn1 -- Series  Load61/RConn1 -- Ground68/LConn1 -- Series  Load64/RConn1
  Series  Load79/RConn1 -- Ground40/LConn1 -- Series  Load77/RConn1 -- Series  Load76/RConn1
  Series  Load100/RConn1 -- Ground55/LConn1 -- Series  Load99/RConn1 -- Series  Load98/RConn1
  Series  Load24/RConn1 -- Series  Load22/RConn1 -- Ground8/LConn1 -- Series  Load23/RConn1
  Series  Load8/RConn1 -- Ground3/LConn1 -- Series  Load7/RConn1 -- Series  Load9/RConn1
  IED14A/RConn1 -- Line1132/RConn1 -- Series  Load43/LConn1 -- IED14/LConn1
  IED12A/RConn2 -- Single-Phase Dynamic Load58/RConn1
  IED9/RConn2 -- Single-Phase Dynamic Load51/RConn1
  SSN Interface Block (3ph)1/LConn2 -- Line718A/RConn2
  IED3/RConn1 -- Single-Phase Dynamic Load40/RConn1
  IED8/RConn1 -- Single-Phase Dynamic Load47/RConn1
  Series  Load42/LConn1 -- IED6/RConn3
  Three-Phase Transformer (Two Windings)2/LConn3 -- IED1/RConn3
  IED9/RConn1 -- Single-Phase Dynamic Load50/RConn1
  SSN Interface Block (3ph)1/LConn1 -- Line718A/RConn1
  Series  Load90/LConn1 -- IED5/RConn2
  IED15/LConn3 -- Line1132/LConn3
  IED8/RConn3 -- Single-Phase Dynamic Load49/RConn1
  IED8/RConn2 -- Single-Phase Dynamic Load48/RConn1
  Line718A/RConn3 -- SSN Interface Block (3ph)1/LConn3
  Line775B/LConn3 -- SSN Interface Block (3ph)/RConn3
  Line775B/LConn1 -- SSN Interface Block (3ph)/RConn1
  SSN Interface Block (3ph)1/RConn2 -- Line718B/LConn2
  IED15/LConn2 -- Line1132/LConn2
  IED2A/RConn3 -- Single-Phase Dynamic Load46/RConn1
  IED10/LConn1 -- Single-Phase Dynamic Load54/RConn1
  Line775B/LConn2 -- SSN Interface Block (3ph)/RConn2
  Line1132/RConn3 -- IED14/LConn3
  Line775A/RConn2 -- SSN Interface Block (3ph)/LConn2
  Line775A/RConn1 -- SSN Interface Block (3ph)/LConn1
  Line775A/RConn3 -- SSN Interface Block (3ph)/LConn3
  IED10/RConn1 -- Series  Load73/LConn1 -- Line614/RConn1
  Ground14/LConn1 -- Series  Load73/RConn1
  SSN Interface Block (3ph)1/RConn1 -- Line718B/LConn1
  IED15/LConn1 -- Line1132/LConn1
  IED12A/RConn3 -- Single-Phase Dynamic Load59/RConn1
  IED13/RConn1 -- Line809/RConn1
  SSN Interface Block (3ph)1/RConn3 -- Line718B/LConn3
  IED12A/RConn1 -- Single-Phase Dynamic Load57/RConn1
  IED13/RConn2 -- Line809/RConn2
  Series  Load88/LConn1 -- IED5/RConn3
  Series  Load83/LConn1 -- IED2/RConn2
  IED13A/RConn1 -- Single-Phase Dynamic Load34/RConn1
  Line1132/RConn2 -- IED14/LConn2
  IED6A/RConn2 -- Single-Phase Dynamic Load38/RConn1
  IED12/RConn1 -- Series  Load92/LConn1
  IED13A/RConn2 -- Single-Phase Dynamic Load35/RConn1
  IED5A/RConn1 -- Single-Phase Dynamic Load60/RConn1
  IED14/RConn1 -- Line937/LConn1
  Series  Load84/LConn1 -- IED7/RConn3
  Series  Load81/LConn1 -- IED2/RConn3
  Series  Load87/LConn1 -- IED7/RConn2
  IED5/RConn1 -- Series  Load89/LConn1
  IED2A/RConn2 -- Single-Phase Dynamic Load45/RConn1
  IED13A/RConn3 -- Single-Phase Dynamic Load36/RConn1
  Line937/LConn2 -- IED14/RConn2
  IED6A/RConn3 -- Single-Phase Dynamic Load39/RConn1
  Series  Load80/LConn1 -- IED6/RConn2
  IED6/RConn1 -- Series  Load60/LConn1
  IED2/RConn1 -- Series  Load82/LConn1
  IED9/RConn3 -- Single-Phase Dynamic Load52/RConn1
  IED14/RConn3 -- Line937/LConn3
  IED5A/RConn3 -- Single-Phase Dynamic Load33/RConn1
  IED13/RConn3 -- Line809/RConn3
  IED3/RConn2 -- Single-Phase Dynamic Load41/RConn1
  IED2A/RConn1 -- Single-Phase Dynamic Load44/RConn1
  IED7/RConn1 -- Series  Load85/LConn1
  IED5A/RConn2 -- Single-Phase Dynamic Load32/RConn1
  Three-Phase Transformer (Two Windings)2/LConn2 -- IED1/RConn2
  IED6A/RConn1 -- Single-Phase Dynamic Load37/RConn1
  IED14A/LConn1 -- Single-Phase Dynamic Load53/RConn1
  Series  Load93/LConn1 -- IED12/RConn2
  IED3/RConn3 -- Single-Phase Dynamic Load43/RConn1
  Single-Phase Dynamic Load30/RConn1 -- IED4/RConn1
  IED7A/LConn1 -- Single-Phase Dynamic Load55/RConn1
  Line405B/LConn3 -- SSN Interface Block (3ph)2/RConn3
  Line405A/RConn3 -- SSN Interface Block (3ph)2/LConn3
  IED11/RConn3 -- PV11/RConn3
  IED11/RConn1 -- PV11/RConn1
  IED11/RConn2 -- PV11/RConn2
  Line405B/LConn2 -- SSN Interface Block (3ph)2/RConn2
  IED4/RConn2 -- Single-Phase Dynamic Load42/RConn1
  Line405A/RConn2 -- SSN Interface Block (3ph)2/LConn2
  Series  Load91/LConn1 -- IED12/RConn3
  Three-Phase Transformer (Two Windings)2/LConn1 -- IED1/RConn1
  Line405B/LConn1 -- SSN Interface Block (3ph)2/RConn1
  IED4/RConn3 -- Single-Phase Dynamic Load56/RConn1
  Ground69/LConn1 -- Series  Load43/RConn1
  Line405A/RConn1 -- SSN Interface Block (3ph)2/LConn1
  Three-Phase Source1/RConn1 -- IED1/LConn1
  Three-Phase Source1/RConn2 -- IED1/LConn2
  Three-Phase Source1/RConn3 -- IED1/LConn3
  Subsystem/LConn1 -- Three-Phase Transformer (Two Windings)2/RConn1
  Three-Phase Transformer (Two Windings)2/RConn2 -- Subsystem/LConn2
  Three-Phase Transformer (Two Windings)2/RConn3 -- Subsystem/LConn3
  Subsystem/RConn3 -- IED15/RConn3
  Subsystem/RConn2 -- IED15/RConn2
  Subsystem/RConn1 -- IED15/RConn1
